simulink model "Adjustedtransfer"  (R2022a)
settings: Solver=VariableStepAuto  StartTime=0.0  StopTime=1e7  RelTol=1e-3
undefined symbols (not defined in the file): denAdjdelay, denAdjZdelay, numAdjdelay, numAdjZdelay, sigbuilder_block
libraries: cstblocks x30, slpidlib x17, slctrlblks x2
(part 1 of 2)
settings Model: Creator=emiel  LastModifiedBy=emiel
settings SolverCC: ZeroCrossAlgorithm=Adaptive
settings DebuggingCC: IgnoredZcDiagnostic=none

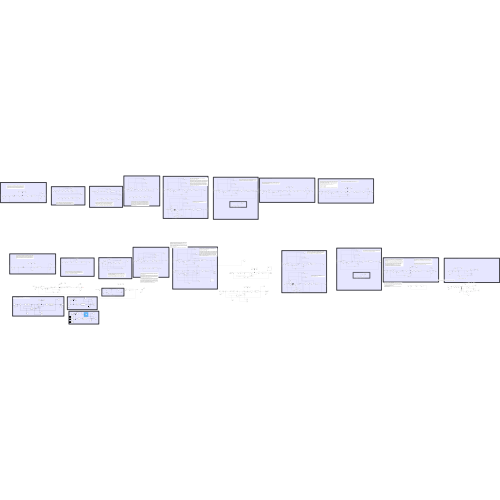
[thumbnail: Simulink's stored preview of the top-level diagram]
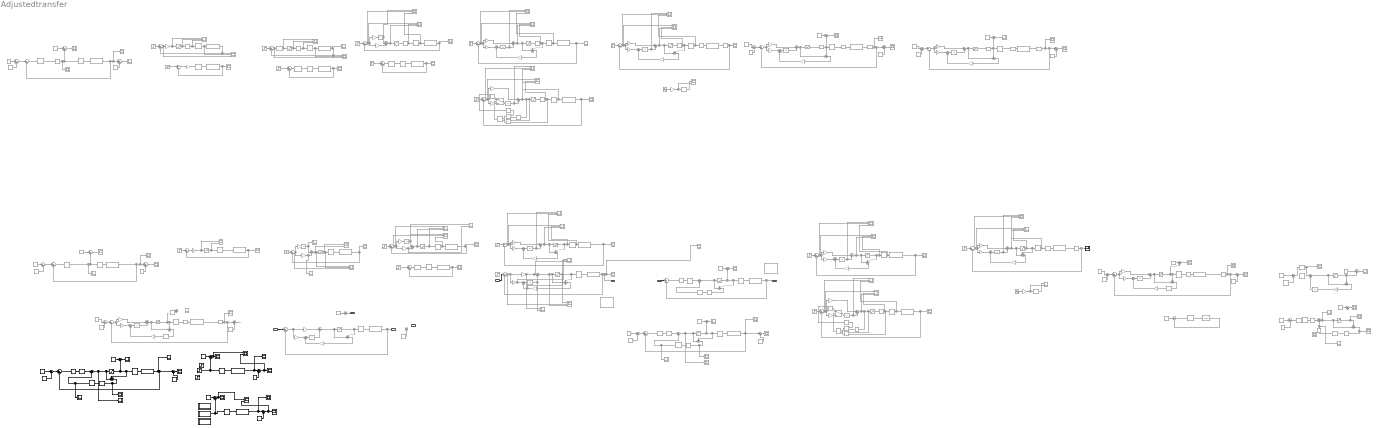
== system Adjustedtransfer ==
  note: sample tijd = 172800 ( 2 dagen) Ki en Kt = 0 en dan ziegler, Kcr = 2,31 Pcr = 347630s
      | --> Kp =  1,03, Ki = 0,00000359 en Kt = 0,00189
  note: Advise mode, een keer -0.0247
  note: Advise mode discrete controller
  note: Controller
  note: Dus als Tfruitref = -1,75 dan zijn we 56000s op -2 --> dit gebruiken als drempel voor max tijd op -2. En als we Tfruitref op -1 dan is het 7800s,
      |
      | Dus een andere vraag is "hoelang moet het groter zijn dan -2 eerdat we zeggen dat we safe zijn? Want als we zeggen, vanaf de eerste keer dat ge boven -2 zit dan kan het door fluctuaties ofzo dat ge ja toch nie oke zit.
      | 	Ge kunt beter teveel dan te weinig pakken hier.
      | Pak dat we 1800s pakken das dan 30 min, dan kunnen we wel veronderstellen dat het wel hoger dan -2 zal blijven
  note: Hier moet dan ook met discrete I controller
  note: Hier moet eigenlijk nog een schema tussen waar ik alles vervang door discrete PI controller, discrete I controller ipv die hold en ook al in de structuur die werkt voor de PLC
  note: Nog zeker eens uitzoeken wat de "responsiviteit" van een koelcel bepaald. En aangeven dat wss het opwarmen een andere snelheid heeft dan het afkoelen, en daardoor is een transferfunctie niet de optimale keuze eigelijk. Dus zou ge in dat geval non lineair moeten gaan. Maar das ja intens ma dat wel aanhalen als ja "issue"
  note: Als we naar Ts kijken zien we dan dat we 8u <-1,5 zitten. Wat opzich nog oke is. qua piekbelaasting. We zien wel dat, dde settling Ts kleiner is dan -1,025 is, da is nie veel verschil met -1 dus in de echte situatie gaan we waarchijnlijk dan nog niet op erorr = 0 zijn. Maar daarvoor dient de I actie uiteindelijk die er dan voor gaat zorgen dat da toch = 0 wodt.
  note: Dus net zeiden we de I actie wat leger voor onstabiliteit op te heffen en de P actie wat lager voor de vibraties/oscilaties op het einde. Dus we doen dan I op 0.000136 en Kt op wortel(0.000136). En we zullen dan Kp blijven verlagen vanaf 33,4 tot we een decent resultaat hebben. En vanaf Kp = 11 en Ki = 0.000136 is het goed stabiel, hebben een beetje overshoot en op het begin war vreemd maar oke nog.
      |
      | Maar als we naar U kijken zien we dat deze van +2 naar -1 gaat en das nie chill, willen liefst dat U gewoon + wordt en dan geleidelijk daalt. En we zien dat de I actie in het begin heel negatief is, dus dat wil zeggen dat Kt dan een grote invloed heeft. Dus oftewel zullen we Ki verlagen oftewel Kt of allebei.
      |
      | Als we naar de anti windup kijken zien we dat deze vooral in het begin moet werken
  note: Als we de waarde Kp en de Ki toepassen zien we dat we in beide gevallen (met en zonder satur) een onstabiel systeem hebben met veel oscilaties. Vreemd aangezien met enkel de P actie het net wel best stabiel was, dus dat wil dan zeggen dat het toevoegen van de I actie voor onstabiliteiten zorgt.
      |
      | En juist ja als we deze verlagen naar 0.000136 of nog eens /10 is het praktisch giga stabiel. Met wel een beetje oscilaties. Maar laten we toch hier eens dieper op ingaan.
  note: Eens bekijken hoelan we dan onder de -1,5 zitten want das wel lage T. exact tot 1e05 dan zitten we terug op -1,5. dus da is dan 1e05*0,8/3600 = 22u13min, da is niet kort dat is wel lang maar bij inkoelen doen ze soms 2 dagen @-2 dus het is niet onmogelijk
  note: We zien dat de P actie in het begin heel negatief is en de I actie cava positief en dan erna is de P actie cava positief en de I cava negatief, waardoor U (de som) positief wordt. Maar we willen juist een negatieve U, dus proberen om de Kp te verlagen 7,74-->5 creëren nog meer overshoot dus miss 7,74 --> 10 nu hebben we inderdaad minder overshoot als we naar Kp = 15 gaan dan is het wel mooi eigelijk
      |
      | Ongeveer idem effect hebben we als we I actie van ....e-05 naar ....e-07 (Kp = 7,74), maar dan gaat uw settling time giga toenemen. dus das ook nie chill.
      |
      | conclu Kp = 15 en Ki en Kt idem
      |
      | Kt veranderen --> instabiliteiten
      |
      | ma tegenover welke kost moeten ook miss eens kijken naar hoelang we dan op -2 zitten.
  note: Tfruit real implementeren --> terug naar het tweaken
  note: Template control schema
  note: testen van de ZOH functie
  note: Discretiseren sws ZOH willen dat de Tset en Tfruit constant blijft totdat we nieuwe T hebben. En omdat ons systeem zo traag is dan boeit da eigenlijk echt nie die discretisatie, als we ZOH op 1 zetten (0,8s) dan is het al zeker snel genoeg en pieter zegt 5ms is de cycle tijd dus zeker oke. Onze PC is eigenlijk sneller dan het systeem.
  note: Dus als we Kp = 7.74 en Ki = ....e-05 en dan Kt = wortel(...e-05) dan gaan we gekke oscilaties hebben. Maar als ik dan Kt/10 doe dan heb ik een perfect signaal.
      | Nog wel uitzoeken hoezo dat daardoor komt.µ
      |
      | Kp = 7.74, Ki= ....e-05, Kt = .....0.0045
      | Dus we zien dat de I en de P actie veel oscilaties hebben, (we zien ook dat voor saturatie en na saturatie idem is). Opmerkelijk is, is dat de P actie bena het spiegelbeeld is van de I actie, waardoor de som van de twee (de U praktisch) veel minder oscilaties hebben. We zien ook dat de I actie in het begin negatief is en dan op het einde meer positief, wat wil zeggen dat er in het begin veel saturatie optreedt en dus in het begin Kt veel moet werken. Maar in het begin willen we juist een positieve U, dus de I actie gaat eigelijk de foute kant op in het begin (doordat er saturatie is) Dus laten we dan Kt wat verlagen waardoor we de I actie in het begin minder negatief gaan maken. --> Kt = 0.00045
      | --> solved --> terugkoppelen naar de vereisten. en ook checken van step van 0-->-1 want das dalen van T en van 0-->1 is stijgen van T
  note: Implementeren van Anti-windup
  note: Simulatie van clamp wilt nie runnen en PID blok houdt geen rekening
      | met rate saturatie. Dus moeten sws handmatig doen
      | maar back caluclation is zo mooi
  note: Bewijzen dat Anti windup nodig is.
  note: Als we de Kp = 0 nemen en de Ki = ....e-07 dan zien we duidelijk dat er anti windup optreedt. Dus dit moeten we sws implementeren. We kunnen discusiëren dat als we de I actie klein genoeg nemen en de Kp niet te groot we een stabiel systeem hebben zonder dat er anti windup nodig is. Maar ten eerste ben ik niet content met dat laatste systeem, de Ess is idd = 0 maar er zijn wel wat oscilaties en overshoot en das nie chill. Ten tweede hebben we hier 1 specifieke koelcel gemodelleert. Als we een andere koelcel nemen bijvoorbeeld en daar zal er wel wind up optreden zijn we in de problemen. Ten derde de totale command is blokkerig, opeens opwarmen dan afkoelene etc. Dus we gaan eens Anti-windup implementeren
  note: Juiste Kp en Ki vinden om stabiel systeem te hebben met saturatie
  note: Als we de waarde van hierlangs toepassen dan zien we dat we een zeer stabiel systeem hebben als we geen saturatie toepassen maar een heel onstabiel als we dat wel doen. De gain is niet te hoog, laten we eens uitproberen wat het verhogen/verlagen van de I actie en de Kp als invloed heeft. Verlagen/ verhogen Kp --> (3,10,15,30) nog altijd zeer onstabiel. Verhogen Ki -->(...e-01 en ....e-03) nog altijd zeer onstabiel. Maar verlagen --> ....e-07 opeens enorm stabiel. Dus dat wil zeggen dat de I actie voor onstabiliteit zorgt.
      |
      | Hoe komt dit? --> groote I actie bekijken in alle gevallen, wss gaat er wind up optreden.
  note: Stap 1: Saturatie toevoegen.
  note: Voor deze loop was de Kcr = 73.4, maar als we de saturatie meegeven, zie hierboven zien we eigenlijk dat we op een veel lagere Kcr naar randstabiel gaan, namenlijk op 17.2 met een Pcr = 458009. Dus als we daarmee dan Ziegler nicholas toepassen krijgen we Kp = 7.74 en Ti = 3.8167e05 --> Ki = 2.0279e-05. Eens kijken wat dat geeft voor stabiliteit zonder dat we saturatie toepassen en zonder dat we anti windup toepassen?
  note: Dus dit is ons standaard model, We hebben telkens de deltaT en de deltaS gemodelleert. Dus we gaan dat ook zo in het model steken. Dus voordat we kunnen beginnen aan de PI regeling moeten we eigelijk 1 ding sws doen en liefst 2. Ten eerste moeten we de Tfruit0 en de Tset0 opmeten dat moet =! moeilijk. Gewoon de koelcel eerst opzetten en dan kijken wat het is. En dan liefst ook een step response doen en dan de parameters per koelcel bepalen voor de plant tf, maar ja als we ervan uitgaan dat da beetje oke is overal cava
  note: Discretiseren
  note: Gaan nu eigelijk terug de fruit en de set temperatuur eraan koppelen. En we zien eigenlijk dat we toch 0,1 graden undershoot hebben als we -1 fruit T willen, dus da is wel nie zo nice. Dus we gaan terug dit huidig systeem moeten analyseren om te kijken of we toch geen parameters moeten tweaken
  note: terug naar het tweaken -->
  note: Template control schema
  note: Discretiseren sws ZOH willen dat de Tset en Tfruit constant blijft totdat we nieuwe T hebben. En omdat ons systeem zo traag is dan boeit da eigenlijk echt nie die discretisatie, als we ZOH op 1s zetten dan is het al zeker snel genoeg en pieter zegt 5ms is de cycle tijd dus zeker oke. Onze PC is eigenlijk sneller dan het systeem.
  note: Implementeren van Anti-windup
  note: Bewijzen dat Anti windup nodig is.
  note: Dus als we Kp = 7.74 en Ki = ....e-05 en dan Kt = wortel(...e-05) dan gaan we gekke oscilaties hebben. Maar als ik dan Kt/10 doe dan heb ik een perfect signaal.
      | Nog wel uitzoeken hoezo dat daardoor komt.µ
      |
      | Kp = 7.74, Ki= ....e-05, Kt = .....0.0045
      | Dus we zien dat de I en de P actie veel oscilaties hebben, (we zien ook dat voor saturatie en na saturatie idem is). Opmerkelijk is, is dat de P actie bena het spiegelbeeld is van de I actie, waardoor de som van de twee (de U praktisch) veel minder oscilaties hebben. We zien ook dat de I actie in het begin negatief is en dan op het einde meer positief, wat wil zeggen dat er in het begin veel saturatie optreedt en dus in het begin Kt veel moet werken. Maar in het begin willen we juist een positieve U, dus de I actie gaat eigelijk de foute kant op in het begin (doordat er saturatie is) Dus laten we dan Kt wat verlagen waardoor we de I actie in het begin minder negatief gaan maken. --> Kt = 0.00045
      | --> solved --> terugkoppelen naar de vereisten. en ook checken van step van 0-->-1 want das dalen van T en van 0-->1 is stijgen van T
  note: Als we de Kp = 33.84 nemen en de Ki = 0.00136 dan zien we dat het systeem onstabiel is en duidelijk dat er anti windup optreedt. De I actie is gewoon giga in vergelijking met de error en de P actie. De I actie is ook max als de P actie 0 is, dus als de error 0 is. Dus anti-windup implementeren.
      |
      | Als we Ki = 0.000136 zien we dat het inderdaad stabieler maar. I actie oscileert wel al niet meer wat goed is, wat wil zeggen dat er eigenlijk geen anti windup nodig is. Dus delta T heef wel wat oscilaties --> U ook --> P ook --> error ook. Dus enkel de P actie heeft wat oscilaties, als we deze nu verlagen naar 12 of 15 hebben we minder kleine oscilaties maar meer grote/overshoot terug dus dat is het ook niet.
      |
      |  We kunnen discusiëren dat als we de I actie klein genoeg nemen en de Kp niet te groot we een stabiel systeem hebben zonder dat er anti windup nodig is. Maar ten eerste ben ik niet content met dat laatste systeem, de Ess is idd = 0 maar er zijn wel wat oscilaties en overshoot en das nie chill. Ten tweede hebben we hier 1 specifieke koelcel gemodelleert. Als we een andere koelcel nemen bijvoorbeeld en daar zal er wel wind up optreden zijn we in de problemen. Ten derde de totale command is blokkerig, opeens opwarmen dan afkoelene etc. Dus we gaan eens Anti-windup implementeren.
      |
      | Maar de P actie moet inderdaad lager om de kleine oscilaties op te lossen
  note: Tfruit real implementeren --> terug naar het tweaken
  note: Stap 1: Saturatie toevoegen.
  note: testen van de ZOH functie
  note: Dus dit is ons standaard model, We hebben telkens de deltaT en de deltaS gemodelleert. Dus we gaan dat ook zo in het model steken. Dus voordat we kunnen beginnen aan de PI regeling moeten we eigelijk 1 ding sws doen en liefst 2. Ten eerste moeten we de Tfruit0 en de Tset0 opmeten dat moet =! moeilijk. Gewoon de koelcel eerst opzetten en dan kijken wat het is. En dan liefst ook een step response doen en dan de parameters per koelcel bepalen voor de plant tf, maar ja als we ervan uitgaan dat da beetje oke is overal cava
  note: Discretiseren
  note: Gaan nu eigelijk terug de fruit en de set temperatuur eraan koppelen. En we een vreemde bult hebben in de rise, Als we dan naar de P,I en U kijken zien we dat dit door de P actie komt, dus deze nog eens verlagen van 7 naar 5 -->totaal niet de bedoeling krijgen nog gekkere bult. Verhogen naar 9 --> weinig effect op de bult, de settling time gaat alleen maar stijgen.
      |
      | I actie verhogen *10 --> bult is weg maar veel oscilatis, dus miss *5 idd minder oscilaties. *3? als we dan *2 of *3 doen hebben we terug die bult Dus miss meer oscilaties maken door I*4 en dan de Kp ook verhogen naar 10 of 15 en zien dan dat da perfect is. Hoe hoger Kp hoe groter de settling time is. Maar als ge lager dan 7 gaat met Kp dan oscilaties. Dus Kp = 12 is goeie compromis
      | xxxxxxxxxxxxxxxxxxxxxxxxxxxxxxxxxxxxxxxxxxxxxxxxxxxxxxxxxxxxxxxxxxxx
      | xxxxxxxxxxxxxxxxx--> Ki = 0,000436 en Kp = 12 en Kt = 0.01166xxxxxxxxxxx
      | xxxxxxxxxxxxxxxxxxxxxxxxxxxxxxxxxxxxxxxxxxxxxxxxxxxxxxxxxxxxxxxxxxxx
  note: Juiste Kp en Ki vinden om stabiel systeem te hebben met saturatie
  note: Voor deze loop was de Kcr = 73.4 (Kp = 33.44), maar als we de saturatie meegeven, zie hierboven zien we eigenlijk dat we op een iets hogere Kcr randstabiel gaan Kcr = 75,2 met een Pcr = 29881 . Dus als we daarmee dan Ziegler nicholas toepassen krijgen we Kp = 33.84 en --> Ki = 0.00136. Eens kijken wat dat geeft voor stabiliteit zonder dat we saturatie toepassen en zonder dat we anti windup toepassen?
  note: Oke hebben dus Kp = 11, Ki = 0.000136 en Kt = wortel(0.000136). Laten we eens kijken wat er gebeurt als we Kt/10 doen --> weinig effect op vibraties, dus terug Kt op normale en Ki/10. Systeem is nu mooi overdempt wat echt goed is. Enkle opnieuw vibraties in de P actie, nog eens verlagen dan? En dan Kp = 7 is ech wat we willen. Overdempt, U verandert niet teveel dus ideaal --> Kp = 7, Ki = 0.0000136n Kt = 0.01166
  note: Simulatie van clamp wilt nie runnen en PID blok houdt geen rekening
      | met rate saturatie. Dus moeten sws handmatig doen
      | maar back caluclation is zo mooi
  note: Implementeren van Anti-windup
  note: Schema maken om twicat te testen. Hadden net 3e6 als tijd
  note: Advise mode, -2 en dan nominaal, als we 89000s op -2°C dan zijn we op fruit T = -1.
      | Dus hebben zolang -2 gezet en dan -0.0247
  Input continious : Inport
  Input : Inport  Port=2
  Input discrete : Inport  Port=3
  -1.5°C : Subsystem  Tag=STV Subsys  LoadFcn=sigbuilder_block('load');  StartFcn=sigbuilder_block('start');  StopFcn=sigbuilder_block('stop');  ClipboardFcn=sigbuilder_block('clipboard');  mask(Sigbuilder block){tuvar=[0:10]}
      mask help: Simulink:masks:SigbuilderBlock_MD
      mask init:
      | if ~strcmp(get_param(bdroot(gcbh),'SimulationStatus'),'stopped') tuvar = sigbuilder_block('maskInit'); end
      settings: CopyFcn=sigbuilder_block('copy');  DeleteFcn=sigbuilder_block('delete');  ModelCloseFcn=sigbuilder_block('modelClose');  PreSaveFcn=sigbuilder_block('preSave');  PauseFcn=sigbuilder_block('pause');  ContinueFcn=sigbuilder_block('continue');  NameChangeFcn=sigbuilder_block('namechange');  OpenFcn=sigbuilder_block('open',[5.5 30 949 418 ]);  CloseFcn=sigbuilder_block('close');
      mask Display: plot(0, 0, 100, 100,[2, 2, 32, 32, 2], [68, 8, 8, 68, 68],[32, 2], [38, 38], [32, 19, 2],[53, 60, 44], [32, 17, 17, 2],[16, 16, 31, 31]);txt = getActiveGroup(gcbh);text(2, 100, txt,'verticalAlignment', 'top');
  -1.75°C1 : Subsystem  Tag=STV Subsys  LoadFcn=sigbuilder_block('load');  StartFcn=sigbuilder_block('start');  StopFcn=sigbuilder_block('stop');  ClipboardFcn=sigbuilder_block('clipboard');  mask(Sigbuilder block){tuvar=[0:10]}
      mask help: Simulink:masks:SigbuilderBlock_MD
      mask init:
      | if ~strcmp(get_param(bdroot(gcbh),'SimulationStatus'),'stopped') tuvar = sigbuilder_block('maskInit'); end
      settings: CopyFcn=sigbuilder_block('copy');  DeleteFcn=sigbuilder_block('delete');  ModelCloseFcn=sigbuilder_block('modelClose');  PreSaveFcn=sigbuilder_block('preSave');  PauseFcn=sigbuilder_block('pause');  ContinueFcn=sigbuilder_block('continue');  NameChangeFcn=sigbuilder_block('namechange');  OpenFcn=sigbuilder_block('open',[5.5 30 949 418 ]);  CloseFcn=sigbuilder_block('close');
      mask Display: plot(0, 0, 100, 100,[2, 2, 32, 32, 2], [68, 8, 8, 68, 68],[32, 2], [38, 38], [32, 19, 2],[53, 60, 44], [32, 17, 17, 2],[16, 16, 31, 31]);txt = getActiveGroup(gcbh);text(2, 100, txt,'verticalAlignment', 'top');
  -2°C : Subsystem  Tag=STV Subsys  LoadFcn=sigbuilder_block('load');  StartFcn=sigbuilder_block('start');  StopFcn=sigbuilder_block('stop');  ClipboardFcn=sigbuilder_block('clipboard');  mask(Sigbuilder block){tuvar=[0:10]}
      mask help: Simulink:masks:SigbuilderBlock_MD
      mask init:
      | if ~strcmp(get_param(bdroot(gcbh),'SimulationStatus'),'stopped') tuvar = sigbuilder_block('maskInit'); end
      settings: CopyFcn=sigbuilder_block('copy');  DeleteFcn=sigbuilder_block('delete');  ModelCloseFcn=sigbuilder_block('modelClose');  PreSaveFcn=sigbuilder_block('preSave');  PauseFcn=sigbuilder_block('pause');  ContinueFcn=sigbuilder_block('continue');  NameChangeFcn=sigbuilder_block('namechange');  OpenFcn=sigbuilder_block('open',[1811 5 949 418 ]);  CloseFcn=sigbuilder_block('close');
      mask Display: plot(0, 0, 100, 100,[2, 2, 32, 32, 2], [68, 8, 8, 68, 68],[32, 2], [38, 38], [32, 19, 2],[53, 60, 44], [32, 17, 17, 2],[16, 16, 31, 31]);txt = getActiveGroup(gcbh);text(2, 100, txt,'verticalAlignment', 'top');
  AND : Logic  Commented=on  IconShape=distinctive  AllPortsSameDT=off  OutDataTypeStr=boolean
  AND2 : Logic  Commented=on  IconShape=distinctive  AllPortsSameDT=off  OutDataTypeStr=boolean
  Anti windup video 2 I actie{,1..6} (7 alike) : Scope  Commented=on  NumInputPorts=3
  Anti windup video 2 I actie clamp : Scope  Commented=on  NumInputPorts=3
  Anti windup video 2 I actie clamp2 : Scope  Commented=on  NumInputPorts=3
  Anti windup video totale command{,1..5,7..9} (9 alike) : Scope  Commented=on  NumInputPorts=3
  Anti-windup Kt : slpidlib/PID Controller  Commented=on  Controller=I  Form=Parallel  TimeDomain=Continuous-time  UseExternalTs=off  SampleTime=-1  IntegratorMethod=Forward Euler  FilterMethod=Forward Euler  ControllerParametersSource=internal  P=1  I=0.000368  UseKiTs=off  D=0  N=100  UseFilter=on  TunerSelectOption=Transfer Function Based (PID Tuner App)  InitialConditionSource=internal  InitialConditionForIntegrator=0  InitialConditionForFilter=0  DifferentiatorICPrevScaledInput=0  ExternalReset=none  TrackingMode=off  Kt=1  LimitOutput=off  SatLimitsSource=internal  UpperSaturationLimit=inf  LowerSaturationLimit=-inf  LinearizeAsGain=off  AntiWindupMode=none  Kb=1  POutMin=[]  POutMax=[]  IOutMin=[]  IOutMax=[]  DOutMin=[]  DOutMax=[]  NOutMin=[]  NOutMax=[]  SumOutMin=[]  SumOutMax=[]  SaturationOutMin=[]  SaturationOutMax=[]  PParamMin=[]  PParamMax=[]  IParamMin=[]  IParamMax=[]  DParamMin=[]  DParamMax=[]  NParamMin=[]  NParamMax=[]  KbParamMin=[]  KbParamMax=[]  KtParamMin=[]  KtParamMax=[]  KbOutMin=[]  KbOutMax=[]  KtOutMin=[]  KtOutMax=[]  IntegratorOutMin=[]  IntegratorOutMax=[]  FilterOutMin=[]  FilterOutMax=[]  SumI1OutMin=[]  SumI1OutMax=[]  SumI2OutMin=[]  SumI2OutMax=[]  SumI3OutMin=[]  SumI3OutMax=[]  SumI4OutMin=[]  SumI4OutMax=[]  SumDOutMin=[]  SumDOutMax=[]  DifferentiatorOutMin=[]  DifferentiatorOutMax=[]  FilterDiffOutCoefMin=[]  FilterDiffOutCoefMax=[]  ReciprocalOutMin=[]  ReciprocalOutMax=[]  SumDenOutMin=[]  SumDenOutMax=[]  SumNumOutMin=[]  SumNumOutMax=[]  DivideOutMin=[]  DivideOutMax=[]  UdiffTsProdOutMin=[]  UdiffTsProdOutMax=[]  NTsProdOutMin=[]  NTsProdOutMax=[]  UintegralTsProdOutMin=[]  UintegralTsProdOutMax=[]  UngainTsProdOutMin=[]  UngainTsProdOutMax=[]  IntegratorContinuousStateAttributes=''  IntegratorStateMustResolveToSignalObject=off  IntegratorRTWStateStorageClass=Auto  FilterContinuousStateAttributes=''  FilterStateMustResolveToSignalObject=off  FilterRTWStateStorageClass=Auto  ParallelPVariant=Disabled  IdealPVariant=Disabled  IVariant=InternalParameters  DVariant=Disabled  IntegratorVariant=Continuous  SatVariant=Disabled  AWVariant=Passthrough  PCopyVariant=Disabled  TRVariant=Disabled  FdbkBlocksVariant=Forward  IdealPFdbkVariant=Disabled  SatFdbkVariant=Disabled  DerivativeFilterVariant=Disabled  NVariant=Disabled  NCopyVariant=Disabled_SignalSpec  FilterICVariant=Disabled  IntegratorICVariant=InternalICs  ExternalResetVariant=Disabled  TRSumVariant=Passthrough  SumFdbkVariant=Disabled  SumVariant=Passthrough_I  TsampFilterVariant=InternalTs  TsampNgainVariant=Passthrough  TsampIntegralVariant=Passthrough  ExternalSaturationOutDataTypeStr=Inherit: Same as second input  aMode=0
  "Anti-windup Kt    " : slpidlib/PID Controller  Commented=on  Controller=I  Form=Parallel  TimeDomain=Continuous-time  UseExternalTs=off  SampleTime=-1  IntegratorMethod=Forward Euler  FilterMethod=Forward Euler  ControllerParametersSource=internal  P=1  I=0.0368  UseKiTs=off  D=0  N=100  UseFilter=on  TunerSelectOption=Transfer Function Based (PID Tuner App)  InitialConditionSource=internal  InitialConditionForIntegrator=0  InitialConditionForFilter=0  DifferentiatorICPrevScaledInput=0  ExternalReset=none  TrackingMode=off  Kt=1  LimitOutput=off  SatLimitsSource=internal  UpperSaturationLimit=inf  LowerSaturationLimit=-inf  LinearizeAsGain=off  AntiWindupMode=none  Kb=1  POutMin=[]  POutMax=[]  IOutMin=[]  IOutMax=[]  DOutMin=[]  DOutMax=[]  NOutMin=[]  NOutMax=[]  SumOutMin=[]  SumOutMax=[]  SaturationOutMin=[]  SaturationOutMax=[]  PParamMin=[]  PParamMax=[]  IParamMin=[]  IParamMax=[]  DParamMin=[]  DParamMax=[]  NParamMin=[]  NParamMax=[]  KbParamMin=[]  KbParamMax=[]  KtParamMin=[]  KtParamMax=[]  KbOutMin=[]  KbOutMax=[]  KtOutMin=[]  KtOutMax=[]  IntegratorOutMin=[]  IntegratorOutMax=[]  FilterOutMin=[]  FilterOutMax=[]  SumI1OutMin=[]  SumI1OutMax=[]  SumI2OutMin=[]  SumI2OutMax=[]  SumI3OutMin=[]  SumI3OutMax=[]  SumI4OutMin=[]  SumI4OutMax=[]  SumDOutMin=[]  SumDOutMax=[]  DifferentiatorOutMin=[]  DifferentiatorOutMax=[]  FilterDiffOutCoefMin=[]  FilterDiffOutCoefMax=[]  ReciprocalOutMin=[]  ReciprocalOutMax=[]  SumDenOutMin=[]  SumDenOutMax=[]  SumNumOutMin=[]  SumNumOutMax=[]  DivideOutMin=[]  DivideOutMax=[]  UdiffTsProdOutMin=[]  UdiffTsProdOutMax=[]  NTsProdOutMin=[]  NTsProdOutMax=[]  UintegralTsProdOutMin=[]  UintegralTsProdOutMax=[]  UngainTsProdOutMin=[]  UngainTsProdOutMax=[]  IntegratorContinuousStateAttributes=''  IntegratorStateMustResolveToSignalObject=off  IntegratorRTWStateStorageClass=Auto  FilterContinuousStateAttributes=''  FilterStateMustResolveToSignalObject=off  FilterRTWStateStorageClass=Auto  ParallelPVariant=Disabled  IdealPVariant=Disabled  IVariant=InternalParameters  DVariant=Disabled  IntegratorVariant=Continuous  SatVariant=Disabled  AWVariant=Passthrough  PCopyVariant=Disabled  TRVariant=Disabled  FdbkBlocksVariant=Forward  IdealPFdbkVariant=Disabled  SatFdbkVariant=Disabled  DerivativeFilterVariant=Disabled  NVariant=Disabled  NCopyVariant=Disabled_SignalSpec  FilterICVariant=Disabled  IntegratorICVariant=InternalICs  ExternalResetVariant=Disabled  TRSumVariant=Passthrough  SumFdbkVariant=Disabled  SumVariant=Passthrough_I  TsampFilterVariant=InternalTs  TsampNgainVariant=Passthrough  TsampIntegralVariant=Passthrough  ExternalSaturationOutDataTypeStr=Inherit: Same as second input  aMode=0
  Anti-windup Kt1 : slpidlib/PID Controller  Commented=on  Controller=I  Form=Parallel  TimeDomain=Continuous-time  UseExternalTs=off  SampleTime=-1  IntegratorMethod=Forward Euler  FilterMethod=Forward Euler  ControllerParametersSource=internal  P=1  I=0.000368  UseKiTs=off  D=0  N=100  UseFilter=on  TunerSelectOption=Transfer Function Based (PID Tuner App)  InitialConditionSource=internal  InitialConditionForIntegrator=0  InitialConditionForFilter=0  DifferentiatorICPrevScaledInput=0  ExternalReset=none  TrackingMode=off  Kt=1  LimitOutput=off  SatLimitsSource=internal  UpperSaturationLimit=inf  LowerSaturationLimit=-inf  LinearizeAsGain=off  AntiWindupMode=none  Kb=1  POutMin=[]  POutMax=[]  IOutMin=[]  IOutMax=[]  DOutMin=[]  DOutMax=[]  NOutMin=[]  NOutMax=[]  SumOutMin=[]  SumOutMax=[]  SaturationOutMin=[]  SaturationOutMax=[]  PParamMin=[]  PParamMax=[]  IParamMin=[]  IParamMax=[]  DParamMin=[]  DParamMax=[]  NParamMin=[]  NParamMax=[]  KbParamMin=[]  KbParamMax=[]  KtParamMin=[]  KtParamMax=[]  KbOutMin=[]  KbOutMax=[]  KtOutMin=[]  KtOutMax=[]  IntegratorOutMin=[]  IntegratorOutMax=[]  FilterOutMin=[]  FilterOutMax=[]  SumI1OutMin=[]  SumI1OutMax=[]  SumI2OutMin=[]  SumI2OutMax=[]  SumI3OutMin=[]  SumI3OutMax=[]  SumI4OutMin=[]  SumI4OutMax=[]  SumDOutMin=[]  SumDOutMax=[]  DifferentiatorOutMin=[]  DifferentiatorOutMax=[]  FilterDiffOutCoefMin=[]  FilterDiffOutCoefMax=[]  ReciprocalOutMin=[]  ReciprocalOutMax=[]  SumDenOutMin=[]  SumDenOutMax=[]  SumNumOutMin=[]  SumNumOutMax=[]  DivideOutMin=[]  DivideOutMax=[]  UdiffTsProdOutMin=[]  UdiffTsProdOutMax=[]  NTsProdOutMin=[]  NTsProdOutMax=[]  UintegralTsProdOutMin=[]  UintegralTsProdOutMax=[]  UngainTsProdOutMin=[]  UngainTsProdOutMax=[]  IntegratorContinuousStateAttributes=''  IntegratorStateMustResolveToSignalObject=off  IntegratorRTWStateStorageClass=Auto  FilterContinuousStateAttributes=''  FilterStateMustResolveToSignalObject=off  FilterRTWStateStorageClass=Auto  ParallelPVariant=Disabled  IdealPVariant=Disabled  IVariant=InternalParameters  DVariant=Disabled  IntegratorVariant=Continuous  SatVariant=Disabled  AWVariant=Passthrough  PCopyVariant=Disabled  TRVariant=Disabled  FdbkBlocksVariant=Forward  IdealPFdbkVariant=Disabled  SatFdbkVariant=Disabled  DerivativeFilterVariant=Disabled  NVariant=Disabled  NCopyVariant=Disabled_SignalSpec  FilterICVariant=Disabled  IntegratorICVariant=InternalICs  ExternalResetVariant=Disabled  TRSumVariant=Passthrough  SumFdbkVariant=Disabled  SumVariant=Passthrough_I  TsampFilterVariant=InternalTs  TsampNgainVariant=Passthrough  TsampIntegralVariant=Passthrough  ExternalSaturationOutDataTypeStr=Inherit: Same as second input  aMode=0
  Anti-windup Kt2 : slpidlib/PID Controller  Controller=I  Form=Parallel  TimeDomain=Continuous-time  UseExternalTs=off  SampleTime=-1  IntegratorMethod=Forward Euler  FilterMethod=Forward Euler  ControllerParametersSource=internal  P=1  I=0.0435  UseKiTs=off  D=0  N=100  UseFilter=on  TunerSelectOption=Transfer Function Based (PID Tuner App)  InitialConditionSource=internal  InitialConditionForIntegrator=0  InitialConditionForFilter=0  DifferentiatorICPrevScaledInput=0  ExternalReset=none  TrackingMode=off  Kt=1  LimitOutput=off  SatLimitsSource=internal  UpperSaturationLimit=inf  LowerSaturationLimit=-inf  LinearizeAsGain=off  AntiWindupMode=none  Kb=1  POutMin=[]  POutMax=[]  IOutMin=[]  IOutMax=[]  DOutMin=[]  DOutMax=[]  NOutMin=[]  NOutMax=[]  SumOutMin=[]  SumOutMax=[]  SaturationOutMin=[]  SaturationOutMax=[]  PParamMin=[]  PParamMax=[]  IParamMin=[]  IParamMax=[]  DParamMin=[]  DParamMax=[]  NParamMin=[]  NParamMax=[]  KbParamMin=[]  KbParamMax=[]  KtParamMin=[]  KtParamMax=[]  KbOutMin=[]  KbOutMax=[]  KtOutMin=[]  KtOutMax=[]  IntegratorOutMin=[]  IntegratorOutMax=[]  FilterOutMin=[]  FilterOutMax=[]  SumI1OutMin=[]  SumI1OutMax=[]  SumI2OutMin=[]  SumI2OutMax=[]  SumI3OutMin=[]  SumI3OutMax=[]  SumI4OutMin=[]  SumI4OutMax=[]  SumDOutMin=[]  SumDOutMax=[]  DifferentiatorOutMin=[]  DifferentiatorOutMax=[]  FilterDiffOutCoefMin=[]  FilterDiffOutCoefMax=[]  ReciprocalOutMin=[]  ReciprocalOutMax=[]  SumDenOutMin=[]  SumDenOutMax=[]  SumNumOutMin=[]  SumNumOutMax=[]  DivideOutMin=[]  DivideOutMax=[]  UdiffTsProdOutMin=[]  UdiffTsProdOutMax=[]  NTsProdOutMin=[]  NTsProdOutMax=[]  UintegralTsProdOutMin=[]  UintegralTsProdOutMax=[]  UngainTsProdOutMin=[]  UngainTsProdOutMax=[]  IntegratorContinuousStateAttributes=''  IntegratorStateMustResolveToSignalObject=off  IntegratorRTWStateStorageClass=Auto  FilterContinuousStateAttributes=''  FilterStateMustResolveToSignalObject=off  FilterRTWStateStorageClass=Auto  ParallelPVariant=Disabled  IdealPVariant=Disabled  IVariant=InternalParameters  DVariant=Disabled  IntegratorVariant=Continuous  SatVariant=Disabled  AWVariant=Passthrough  PCopyVariant=Disabled  TRVariant=Disabled  FdbkBlocksVariant=Forward  IdealPFdbkVariant=Disabled  SatFdbkVariant=Disabled  DerivativeFilterVariant=Disabled  NVariant=Disabled  NCopyVariant=Disabled_SignalSpec  FilterICVariant=Disabled  IntegratorICVariant=InternalICs  ExternalResetVariant=Disabled  TRSumVariant=Passthrough  SumFdbkVariant=Disabled  SumVariant=Passthrough_I  TsampFilterVariant=InternalTs  TsampNgainVariant=Passthrough  TsampIntegralVariant=Passthrough  ExternalSaturationOutDataTypeStr=Inherit: Same as second input  aMode=0
  Bias1 : Constant  Commented=on  Value=-1
  Bias2 : Constant  Commented=on  Value=-1
  Bode Plot : slctrlblks/Model Verification/Check Bode  Characteristics  Commented=on  InstantiateOnLoad=on  SaveOperatingPoints=off  LinearizationIOs={'/Plant discrete', 1, 'out', 'on', '';'/Input discrete', 1, 'in', 'on', ''}  LinearizeAt=SnapshotTimes  SnapshotTimes=[0]  TriggerType=rising  SampleTime=auto  RateConversionMethod=zoh  PreWarpFreq=10  UseExactDelayModel=off  UseFullBlockNameLabels=off  UseBusSignalLabels=off  enabled=on  stopWhenAssertionFail=off  export=off  ViewDlgPos=[3.66666666666667 232.333333333333 538.666666666667 390]  OpenViewOnLoad=off  LaunchViewOnOpen=off  FrequencyUnits=rad/s  MagnitudeUnits=dB  PhaseUnits=deg  TimeUnits=seconds  EnableUpperBound=off  UpperBoundFrequencies=[]  UpperBoundMagnitudes=[]  EnableLowerBound=off  LowerBoundFrequencies=[]  LowerBoundMagnitudes=[]
  Bode Plot1 : slctrlblks/Model Verification/Check Bode  Characteristics  Commented=on  InstantiateOnLoad=on  SaveOperatingPoints=off  LinearizationIOs={'/Plant continious', 1, 'out', 'on', '';'/Input continious', 1, 'in', 'on', ''}  LinearizeAt=SnapshotTimes  SnapshotTimes=[0]  TriggerType=rising  SampleTime=auto  RateConversionMethod=zoh  PreWarpFreq=10  UseExactDelayModel=off  UseFullBlockNameLabels=off  UseBusSignalLabels=off  enabled=on  stopWhenAssertionFail=off  export=off  ViewDlgPos=[2151 -28.3333333333333 733.333333333333 528]  OpenViewOnLoad=off  LaunchViewOnOpen=off  FrequencyUnits=rad/s  MagnitudeUnits=dB  PhaseUnits=deg  TimeUnits=seconds  EnableUpperBound=off  UpperBoundFrequencies=[]  UpperBoundMagnitudes=[]  EnableLowerBound=off  LowerBoundFrequencies=[]  LowerBoundMagnitudes=[]
      settings: SaveToWorkspace=on  SaveName=sys2
  Constant{1..4} (4 alike) : Constant  Commented=on  Value=-0.75
  Constant5 : Constant  Commented=on  Value=0
  Constant6 : Constant  Commented=on  Value=-1
  Constant8 : Constant  Commented=on  Value=-1
  Constant9 : Constant  Commented=on  Value=0
  Continious model{,1..3} (4 alike) : Scope  Commented=on
  Delta S : Scope  Commented=on
  Delta S1 : Scope  Commented=on
  Discrete PID Controller : slpidlib/PID Controller  Commented=on  Controller=PI  Form=Parallel  TimeDomain=Discrete-time  UseExternalTs=off  SampleTime=1  IntegratorMethod=Backward Euler  FilterMethod=Backward Euler  ControllerParametersSource=internal  P=12  I=0.0000436  UseKiTs=off  D=0  N=100  UseFilter=on  TunerSelectOption=Transfer Function Based (PID Tuner App)  InitialConditionSource=internal  InitialConditionForIntegrator=0  InitialConditionForFilter=0  DifferentiatorICPrevScaledInput=0  ExternalReset=none  TrackingMode=off  Kt=1  LimitOutput=off  SatLimitsSource=internal  UpperSaturationLimit=inf  LowerSaturationLimit=-inf  LinearizeAsGain=off  AntiWindupMode=none  Kb=1  POutMin=[]  POutMax=[]  IOutMin=[]  IOutMax=[]  DOutMin=[]  DOutMax=[]  NOutMin=[]  NOutMax=[]  SumOutMin=[]  SumOutMax=[]  SaturationOutMin=[]  SaturationOutMax=[]  PParamMin=[]  PParamMax=[]  IParamMin=[]  IParamMax=[]  DParamMin=[]  DParamMax=[]  NParamMin=[]  NParamMax=[]  KbParamMin=[]  KbParamMax=[]  KtParamMin=[]  KtParamMax=[]  KbOutMin=[]  KbOutMax=[]  KtOutMin=[]  KtOutMax=[]  IntegratorOutMin=[]  IntegratorOutMax=[]  FilterOutMin=[]  FilterOutMax=[]  SumI1OutMin=[]  SumI1OutMax=[]  SumI2OutMin=[]  SumI2OutMax=[]  SumI3OutMin=[]  SumI3OutMax=[]  SumI4OutMin=[]  SumI4OutMax=[]  SumDOutMin=[]  SumDOutMax=[]  DifferentiatorOutMin=[]  DifferentiatorOutMax=[]  FilterDiffOutCoefMin=[]  FilterDiffOutCoefMax=[]  ReciprocalOutMin=[]  ReciprocalOutMax=[]  SumDenOutMin=[]  SumDenOutMax=[]  SumNumOutMin=[]  SumNumOutMax=[]  DivideOutMin=[]  DivideOutMax=[]  UdiffTsProdOutMin=[]  UdiffTsProdOutMax=[]  NTsProdOutMin=[]  NTsProdOutMax=[]  UintegralTsProdOutMin=[]  UintegralTsProdOutMax=[]  UngainTsProdOutMin=[]  UngainTsProdOutMax=[]  IntegratorContinuousStateAttributes=''  IntegratorStateMustResolveToSignalObject=off  IntegratorRTWStateStorageClass=Auto  FilterContinuousStateAttributes=''  FilterStateMustResolveToSignalObject=off  FilterRTWStateStorageClass=Auto  ParallelPVariant=InternalParameters  IdealPVariant=Disabled  IVariant=InternalParameters  DVariant=Disabled  IntegratorVariant=Discrete  SatVariant=Disabled  AWVariant=Passthrough  PCopyVariant=Disabled  TRVariant=Disabled  FdbkBlocksVariant=Forward  IdealPFdbkVariant=Disabled  SatFdbkVariant=Disabled  DerivativeFilterVariant=Disabled  NVariant=Disabled  NCopyVariant=Disabled_SignalSpec  FilterICVariant=Disabled  IntegratorICVariant=InternalICs  ExternalResetVariant=Disabled  TRSumVariant=Passthrough  SumFdbkVariant=Disabled  SumVariant=Sum_PI  TsampFilterVariant=InternalTs  TsampNgainVariant=Passthrough  TsampIntegralVariant=Passthrough  ExternalSaturationOutDataTypeStr=Inherit: Same as second input  aMode=0
  Discrete PID Controller1 : slpidlib/PID Controller  Commented=on  Controller=PI  Form=Parallel  TimeDomain=Continuous-time  UseExternalTs=off  SampleTime=1  IntegratorMethod=Backward Euler  FilterMethod=Forward Euler  ControllerParametersSource=internal  P=15  I=0.000136  UseKiTs=off  D=0  N=100  UseFilter=on  TunerSelectOption=Transfer Function Based (PID Tuner App)  InitialConditionSource=internal  InitialConditionForIntegrator=0  InitialConditionForFilter=0  DifferentiatorICPrevScaledInput=0  ExternalReset=none  TrackingMode=off  Kt=1  LimitOutput=off  SatLimitsSource=internal  UpperSaturationLimit=inf  LowerSaturationLimit=-inf  LinearizeAsGain=off  AntiWindupMode=none  Kb=1  POutMin=[]  POutMax=[]  IOutMin=[]  IOutMax=[]  DOutMin=[]  DOutMax=[]  NOutMin=[]  NOutMax=[]  SumOutMin=[]  SumOutMax=[]  SaturationOutMin=[]  SaturationOutMax=[]  PParamMin=[]  PParamMax=[]  IParamMin=[]  IParamMax=[]  DParamMin=[]  DParamMax=[]  NParamMin=[]  NParamMax=[]  KbParamMin=[]  KbParamMax=[]  KtParamMin=[]  KtParamMax=[]  KbOutMin=[]  KbOutMax=[]  KtOutMin=[]  KtOutMax=[]  IntegratorOutMin=[]  IntegratorOutMax=[]  FilterOutMin=[]  FilterOutMax=[]  SumI1OutMin=[]  SumI1OutMax=[]  SumI2OutMin=[]  SumI2OutMax=[]  SumI3OutMin=[]  SumI3OutMax=[]  SumI4OutMin=[]  SumI4OutMax=[]  SumDOutMin=[]  SumDOutMax=[]  DifferentiatorOutMin=[]  DifferentiatorOutMax=[]  FilterDiffOutCoefMin=[]  FilterDiffOutCoefMax=[]  ReciprocalOutMin=[]  ReciprocalOutMax=[]  SumDenOutMin=[]  SumDenOutMax=[]  SumNumOutMin=[]  SumNumOutMax=[]  DivideOutMin=[]  DivideOutMax=[]  UdiffTsProdOutMin=[]  UdiffTsProdOutMax=[]  NTsProdOutMin=[]  NTsProdOutMax=[]  UintegralTsProdOutMin=[]  UintegralTsProdOutMax=[]  UngainTsProdOutMin=[]  UngainTsProdOutMax=[]  IntegratorContinuousStateAttributes=''  IntegratorStateMustResolveToSignalObject=off  IntegratorRTWStateStorageClass=Auto  FilterContinuousStateAttributes=''  FilterStateMustResolveToSignalObject=off  FilterRTWStateStorageClass=Auto  ParallelPVariant=InternalParameters  IdealPVariant=Disabled  IVariant=InternalParameters  DVariant=Disabled  IntegratorVariant=Continuous  SatVariant=Disabled  AWVariant=Passthrough  PCopyVariant=Disabled  TRVariant=Disabled  FdbkBlocksVariant=Forward  IdealPFdbkVariant=Disabled  SatFdbkVariant=Disabled  DerivativeFilterVariant=Disabled  NVariant=Disabled  NCopyVariant=Disabled_SignalSpec  FilterICVariant=Disabled  IntegratorICVariant=InternalICs  ExternalResetVariant=Disabled  TRSumVariant=Passthrough  SumFdbkVariant=Disabled  SumVariant=Sum_PI  TsampFilterVariant=InternalTs  TsampNgainVariant=Passthrough  TsampIntegralVariant=Passthrough  ExternalSaturationOutDataTypeStr=Inherit: Same as second input  aMode=0
  Discrete PID Controller2 : slpidlib/PID Controller  Commented=on  Controller=PI  Form=Parallel  TimeDomain=Continuous-time  UseExternalTs=off  SampleTime=1  IntegratorMethod=Backward Euler  FilterMethod=Forward Euler  ControllerParametersSource=internal  P=15  I=0.0136  UseKiTs=off  D=0  N=100  UseFilter=on  TunerSelectOption=Transfer Function Based (PID Tuner App)  InitialConditionSource=internal  InitialConditionForIntegrator=0  InitialConditionForFilter=0  DifferentiatorICPrevScaledInput=0  ExternalReset=none  TrackingMode=off  Kt=1  LimitOutput=off  SatLimitsSource=internal  UpperSaturationLimit=inf  LowerSaturationLimit=-inf  LinearizeAsGain=off  AntiWindupMode=none  Kb=1  POutMin=[]  POutMax=[]  IOutMin=[]  IOutMax=[]  DOutMin=[]  DOutMax=[]  NOutMin=[]  NOutMax=[]  SumOutMin=[]  SumOutMax=[]  SaturationOutMin=[]  SaturationOutMax=[]  PParamMin=[]  PParamMax=[]  IParamMin=[]  IParamMax=[]  DParamMin=[]  DParamMax=[]  NParamMin=[]  NParamMax=[]  KbParamMin=[]  KbParamMax=[]  KtParamMin=[]  KtParamMax=[]  KbOutMin=[]  KbOutMax=[]  KtOutMin=[]  KtOutMax=[]  IntegratorOutMin=[]  IntegratorOutMax=[]  FilterOutMin=[]  FilterOutMax=[]  SumI1OutMin=[]  SumI1OutMax=[]  SumI2OutMin=[]  SumI2OutMax=[]  SumI3OutMin=[]  SumI3OutMax=[]  SumI4OutMin=[]  SumI4OutMax=[]  SumDOutMin=[]  SumDOutMax=[]  DifferentiatorOutMin=[]  DifferentiatorOutMax=[]  FilterDiffOutCoefMin=[]  FilterDiffOutCoefMax=[]  ReciprocalOutMin=[]  ReciprocalOutMax=[]  SumDenOutMin=[]  SumDenOutMax=[]  SumNumOutMin=[]  SumNumOutMax=[]  DivideOutMin=[]  DivideOutMax=[]  UdiffTsProdOutMin=[]  UdiffTsProdOutMax=[]  NTsProdOutMin=[]  NTsProdOutMax=[]  UintegralTsProdOutMin=[]  UintegralTsProdOutMax=[]  UngainTsProdOutMin=[]  UngainTsProdOutMax=[]  IntegratorContinuousStateAttributes=''  IntegratorStateMustResolveToSignalObject=off  IntegratorRTWStateStorageClass=Auto  FilterContinuousStateAttributes=''  FilterStateMustResolveToSignalObject=off  FilterRTWStateStorageClass=Auto  ParallelPVariant=InternalParameters  IdealPVariant=Disabled  IVariant=InternalParameters  DVariant=Disabled  IntegratorVariant=Continuous  SatVariant=Disabled  AWVariant=Passthrough  PCopyVariant=Disabled  TRVariant=Disabled  FdbkBlocksVariant=Forward  IdealPFdbkVariant=Disabled  SatFdbkVariant=Disabled  DerivativeFilterVariant=Disabled  NVariant=Disabled  NCopyVariant=Disabled_SignalSpec  FilterICVariant=Disabled  IntegratorICVariant=InternalICs  ExternalResetVariant=Disabled  TRSumVariant=Passthrough  SumFdbkVariant=Disabled  SumVariant=Sum_PI  TsampFilterVariant=InternalTs  TsampNgainVariant=Passthrough  TsampIntegralVariant=Passthrough  ExternalSaturationOutDataTypeStr=Inherit: Same as second input  aMode=0
  Discrete PID Controller3 : slpidlib/PID Controller  Commented=on  Controller=PI  Form=Parallel  TimeDomain=Continuous-time  UseExternalTs=off  SampleTime=1  IntegratorMethod=Backward Euler  FilterMethod=Forward Euler  ControllerParametersSource=internal  P=15  I=0.000136  UseKiTs=off  D=0  N=100  UseFilter=on  TunerSelectOption=Transfer Function Based (PID Tuner App)  InitialConditionSource=internal  InitialConditionForIntegrator=0  InitialConditionForFilter=0  DifferentiatorICPrevScaledInput=0  ExternalReset=none  TrackingMode=off  Kt=1  LimitOutput=off  SatLimitsSource=internal  UpperSaturationLimit=inf  LowerSaturationLimit=-inf  LinearizeAsGain=off  AntiWindupMode=none  Kb=1  POutMin=[]  POutMax=[]  IOutMin=[]  IOutMax=[]  DOutMin=[]  DOutMax=[]  NOutMin=[]  NOutMax=[]  SumOutMin=[]  SumOutMax=[]  SaturationOutMin=[]  SaturationOutMax=[]  PParamMin=[]  PParamMax=[]  IParamMin=[]  IParamMax=[]  DParamMin=[]  DParamMax=[]  NParamMin=[]  NParamMax=[]  KbParamMin=[]  KbParamMax=[]  KtParamMin=[]  KtParamMax=[]  KbOutMin=[]  KbOutMax=[]  KtOutMin=[]  KtOutMax=[]  IntegratorOutMin=[]  IntegratorOutMax=[]  FilterOutMin=[]  FilterOutMax=[]  SumI1OutMin=[]  SumI1OutMax=[]  SumI2OutMin=[]  SumI2OutMax=[]  SumI3OutMin=[]  SumI3OutMax=[]  SumI4OutMin=[]  SumI4OutMax=[]  SumDOutMin=[]  SumDOutMax=[]  DifferentiatorOutMin=[]  DifferentiatorOutMax=[]  FilterDiffOutCoefMin=[]  FilterDiffOutCoefMax=[]  ReciprocalOutMin=[]  ReciprocalOutMax=[]  SumDenOutMin=[]  SumDenOutMax=[]  SumNumOutMin=[]  SumNumOutMax=[]  DivideOutMin=[]  DivideOutMax=[]  UdiffTsProdOutMin=[]  UdiffTsProdOutMax=[]  NTsProdOutMin=[]  NTsProdOutMax=[]  UintegralTsProdOutMin=[]  UintegralTsProdOutMax=[]  UngainTsProdOutMin=[]  UngainTsProdOutMax=[]  IntegratorContinuousStateAttributes=''  IntegratorStateMustResolveToSignalObject=off  IntegratorRTWStateStorageClass=Auto  FilterContinuousStateAttributes=''  FilterStateMustResolveToSignalObject=off  FilterRTWStateStorageClass=Auto  ParallelPVariant=InternalParameters  IdealPVariant=Disabled  IVariant=InternalParameters  DVariant=Disabled  IntegratorVariant=Continuous  SatVariant=Disabled  AWVariant=Passthrough  PCopyVariant=Disabled  TRVariant=Disabled  FdbkBlocksVariant=Forward  IdealPFdbkVariant=Disabled  SatFdbkVariant=Disabled  DerivativeFilterVariant=Disabled  NVariant=Disabled  NCopyVariant=Disabled_SignalSpec  FilterICVariant=Disabled  IntegratorICVariant=InternalICs  ExternalResetVariant=Disabled  TRSumVariant=Passthrough  SumFdbkVariant=Disabled  SumVariant=Sum_PI  TsampFilterVariant=InternalTs  TsampNgainVariant=Passthrough  TsampIntegralVariant=Passthrough  ExternalSaturationOutDataTypeStr=Inherit: Same as second input  aMode=0
  Discrete PID Controller4 : slpidlib/PID Controller  Controller=PI  Form=Parallel  TimeDomain=Continuous-time  UseExternalTs=off  SampleTime=1  IntegratorMethod=Backward Euler  FilterMethod=Forward Euler  ControllerParametersSource=internal  P=0.5  I=0.000000359  UseKiTs=off  D=0  N=100  UseFilter=on  TunerSelectOption=Transfer Function Based (PID Tuner App)  InitialConditionSource=internal  InitialConditionForIntegrator=0  InitialConditionForFilter=0  DifferentiatorICPrevScaledInput=0  ExternalReset=none  TrackingMode=off  Kt=1  LimitOutput=off  SatLimitsSource=internal  UpperSaturationLimit=inf  LowerSaturationLimit=-inf  LinearizeAsGain=off  AntiWindupMode=none  Kb=1  POutMin=[]  POutMax=[]  IOutMin=[]  IOutMax=[]  DOutMin=[]  DOutMax=[]  NOutMin=[]  NOutMax=[]  SumOutMin=[]  SumOutMax=[]  SaturationOutMin=[]  SaturationOutMax=[]  PParamMin=[]  PParamMax=[]  IParamMin=[]  IParamMax=[]  DParamMin=[]  DParamMax=[]  NParamMin=[]  NParamMax=[]  KbParamMin=[]  KbParamMax=[]  KtParamMin=[]  KtParamMax=[]  KbOutMin=[]  KbOutMax=[]  KtOutMin=[]  KtOutMax=[]  IntegratorOutMin=[]  IntegratorOutMax=[]  FilterOutMin=[]  FilterOutMax=[]  SumI1OutMin=[]  SumI1OutMax=[]  SumI2OutMin=[]  SumI2OutMax=[]  SumI3OutMin=[]  SumI3OutMax=[]  SumI4OutMin=[]  SumI4OutMax=[]  SumDOutMin=[]  SumDOutMax=[]  DifferentiatorOutMin=[]  DifferentiatorOutMax=[]  FilterDiffOutCoefMin=[]  FilterDiffOutCoefMax=[]  ReciprocalOutMin=[]  ReciprocalOutMax=[]  SumDenOutMin=[]  SumDenOutMax=[]  SumNumOutMin=[]  SumNumOutMax=[]  DivideOutMin=[]  DivideOutMax=[]  UdiffTsProdOutMin=[]  UdiffTsProdOutMax=[]  NTsProdOutMin=[]  NTsProdOutMax=[]  UintegralTsProdOutMin=[]  UintegralTsProdOutMax=[]  UngainTsProdOutMin=[]  UngainTsProdOutMax=[]  IntegratorContinuousStateAttributes=''  IntegratorStateMustResolveToSignalObject=off  IntegratorRTWStateStorageClass=Auto  FilterContinuousStateAttributes=''  FilterStateMustResolveToSignalObject=off  FilterRTWStateStorageClass=Auto  ParallelPVariant=InternalParameters  IdealPVariant=Disabled  IVariant=InternalParameters  DVariant=Disabled  IntegratorVariant=Continuous  SatVariant=Disabled  AWVariant=Passthrough  PCopyVariant=Disabled  TRVariant=Disabled  FdbkBlocksVariant=Forward  IdealPFdbkVariant=Disabled  SatFdbkVariant=Disabled  DerivativeFilterVariant=Disabled  NVariant=Disabled  NCopyVariant=Disabled_SignalSpec  FilterICVariant=Disabled  IntegratorICVariant=InternalICs  ExternalResetVariant=Disabled  TRSumVariant=Passthrough  SumFdbkVariant=Disabled  SumVariant=Sum_PI  TsampFilterVariant=InternalTs  TsampNgainVariant=Passthrough  TsampIntegralVariant=Passthrough  ExternalSaturationOutDataTypeStr=Inherit: Same as second input  aMode=0
  Discrete model : Scope  Commented=on
  Discrete model1 : Scope
  Echte Ts : Scope  Commented=on
  Echte Ts1 : Scope  Commented=on
  Equal : RelationalOperator  Commented=on  Operator=~=  OutDataTypeStr=boolean  RndMeth=Simplest  InputSameDT=off
  Equal1 : RelationalOperator  Commented=on  Operator===  OutDataTypeStr=boolean  RndMeth=Simplest  InputSameDT=off
  Equal4 : RelationalOperator  Commented=on  Operator=~=  OutDataTypeStr=boolean  RndMeth=Simplest  InputSameDT=off
  Equal5 : RelationalOperator  Commented=on  Operator===  OutDataTypeStr=boolean  RndMeth=Simplest  InputSameDT=off
  Gain : Gain  Commented=on  Gain=17.2
  Gain1 : Gain  Commented=on  Gain=73.4
  Gain2 : Gain  Commented=on  Gain=5
  Gain3 : Gain  Commented=on  Gain=75.2
  Gain5 : Gain  Commented=on  Gain=5
  Hoeveel Tf veraderen : Scope  Commented=on
  Hoeveel Tf veraderen1 : Scope  Commented=on
  Hold U{,1..6} (7 alike) : ZeroOrderHold  Commented=on
  Hold measurement{1..7} (7 alike) : ZeroOrderHold  Commented=on
  Integrator{,1..16} (17 alike) : Integrator  Commented=on
  Ki : Gain  Commented=on  Gain=2.0279e-07
  "Ki " : Gain  Commented=on  Gain=0.00136
  Ki{1..5,13} (6 alike) : Gain  Commented=on  Gain=2.0279e-05
  Ki10 : Gain  Commented=on  Gain=0.0000436
  Ki11 : Gain  Commented=on  Gain=0.00136
  Ki12 : Gain  Commented=on  Gain=0.0000136
  Ki14 : Gain  Commented=on  Gain=0.0000436
  Ki6 : Gain  Commented=on  Gain=0.000136
  Ki7 : Gain  Commented=on  Gain=0.000136
  Ki8 : Gain  Commented=on  Gain=0.000136
  Ki9 : Gain  Commented=on  Gain=0.0000136
  Kp{,1,3..4} (4 alike) : Gain  Commented=on  Gain=7.74
  "Kp " : Gain  Commented=on  Gain=33.84
  Kp10 : Gain  Commented=on  Gain=12
  Kp11 : Gain  Commented=on  Gain=33.84
  Kp12 : Gain  Commented=on  Gain=7
  Kp13 : Gain  Commented=on
  Kp14 : Gain  Commented=on  Gain=12
  Kp2 : Gain  Commented=on
  Kp5 : Gain  Commented=on  Gain=15
  Kp6 : Gain  Commented=on  Gain=12
  Kp7 : Gain  Commented=on  Gain=11
  Kp8 : Gain  Commented=on  Gain=15
  Kp9 : Gain  Commented=on  Gain=7
  Kt{,1..3} (4 alike) : Gain  Commented=on  Gain=0.00045
  "Kt " : Gain  Commented=on  Gain=0.01166
  Kt{4..8,10} (6 alike) : Gain  Commented=on  Gain=0.01166
  Kt9 : Gain  Commented=on  Gain=0.000368
  OL met saturatie : Scope  Commented=on  NumInputPorts=3
  OL met saturatie 2 : Scope  Commented=on  NumInputPorts=3
  OL zonder saturatie{,1..2,4} (4 alike) : Scope  Commented=on
  PID Controller : slpidlib/PID Controller  Commented=on  Controller=PI  Form=Parallel  TimeDomain=Continuous-time  UseExternalTs=off  SampleTime=-1  IntegratorMethod=Forward Euler  FilterMethod=Forward Euler  ControllerParametersSource=internal  P=12  I=0.0000436  UseKiTs=off  D=0  N=100  UseFilter=on  TunerSelectOption=Transfer Function Based (PID Tuner App)  InitialConditionSource=internal  InitialConditionForIntegrator=0  InitialConditionForFilter=0  DifferentiatorICPrevScaledInput=0  ExternalReset=none  TrackingMode=off  Kt=1  LimitOutput=off  SatLimitsSource=internal  UpperSaturationLimit=inf  LowerSaturationLimit=-inf  LinearizeAsGain=on  AntiWindupMode=none  Kb=1  POutMin=[]  POutMax=[]  IOutMin=[]  IOutMax=[]  DOutMin=[]  DOutMax=[]  NOutMin=[]  NOutMax=[]  SumOutMin=[]  SumOutMax=[]  SaturationOutMin=[]  SaturationOutMax=[]  PParamMin=[]  PParamMax=[]  IParamMin=[]  IParamMax=[]  DParamMin=[]  DParamMax=[]  NParamMin=[]  NParamMax=[]  KbParamMin=[]  KbParamMax=[]  KtParamMin=[]  KtParamMax=[]  KbOutMin=[]  KbOutMax=[]  KtOutMin=[]  KtOutMax=[]  IntegratorOutMin=[]  IntegratorOutMax=[]  FilterOutMin=[]  FilterOutMax=[]  SumI1OutMin=[]  SumI1OutMax=[]  SumI2OutMin=[]  SumI2OutMax=[]  SumI3OutMin=[]  SumI3OutMax=[]  SumI4OutMin=[]  SumI4OutMax=[]  SumDOutMin=[]  SumDOutMax=[]  DifferentiatorOutMin=[]  DifferentiatorOutMax=[]  FilterDiffOutCoefMin=[]  FilterDiffOutCoefMax=[]  ReciprocalOutMin=[]  ReciprocalOutMax=[]  SumDenOutMin=[]  SumDenOutMax=[]  SumNumOutMin=[]  SumNumOutMax=[]  DivideOutMin=[]  DivideOutMax=[]  UdiffTsProdOutMin=[]  UdiffTsProdOutMax=[]  NTsProdOutMin=[]  NTsProdOutMax=[]  UintegralTsProdOutMin=[]  UintegralTsProdOutMax=[]  UngainTsProdOutMin=[]  UngainTsProdOutMax=[]  IntegratorContinuousStateAttributes=''  IntegratorStateMustResolveToSignalObject=off  IntegratorRTWStateStorageClass=Auto  FilterContinuousStateAttributes=''  FilterStateMustResolveToSignalObject=off  FilterRTWStateStorageClass=Auto  ParallelPVariant=InternalParameters  IdealPVariant=Disabled  IVariant=InternalParameters  DVariant=Disabled  IntegratorVariant=Continuous  SatVariant=Disabled  AWVariant=Passthrough  PCopyVariant=Disabled  TRVariant=Disabled  FdbkBlocksVariant=Forward  IdealPFdbkVariant=Disabled  SatFdbkVariant=Disabled  DerivativeFilterVariant=Disabled  NVariant=Disabled  NCopyVariant=Disabled_SignalSpec  FilterICVariant=Disabled  IntegratorICVariant=InternalICs  ExternalResetVariant=Disabled  TRSumVariant=Passthrough  SumFdbkVariant=Disabled  SumVariant=Sum_PI  TsampFilterVariant=InternalTs  TsampNgainVariant=Passthrough  TsampIntegralVariant=Passthrough  ExternalSaturationOutDataTypeStr=Inherit: Same as second input  aMode=0
  PID Controller (Gv)1 : slpidlib/PID Controller  Commented=on  Controller=PI  Form=Parallel  TimeDomain=Continuous-time  UseExternalTs=off  SampleTime=-1  IntegratorMethod=Forward Euler  FilterMethod=Forward Euler  ControllerParametersSource=internal  P=1  I=0  UseKiTs=off  D=0  N=100  UseFilter=on  TunerSelectOption=Transfer Function Based (PID Tuner App)  InitialConditionSource=internal  InitialConditionForIntegrator=0  InitialConditionForFilter=0  DifferentiatorICPrevScaledInput=0  ExternalReset=none  TrackingMode=off  Kt=1  LimitOutput=on  SatLimitsSource=internal  UpperSaturationLimit=2  LowerSaturationLimit=-1  LinearizeAsGain=on  AntiWindupMode=clamping  Kb=1  POutMin=[]  POutMax=[]  IOutMin=[]  IOutMax=[]  DOutMin=[]  DOutMax=[]  NOutMin=[]  NOutMax=[]  SumOutMin=[]  SumOutMax=[]  SaturationOutMin=[]  SaturationOutMax=[]  PParamMin=[]  PParamMax=[]  IParamMin=[]  IParamMax=[]  DParamMin=[]  DParamMax=[]  NParamMin=[]  NParamMax=[]  KbParamMin=[]  KbParamMax=[]  KtParamMin=[]  KtParamMax=[]  KbOutMin=[]  KbOutMax=[]  KtOutMin=[]  KtOutMax=[]  IntegratorOutMin=[]  IntegratorOutMax=[]  FilterOutMin=[]  FilterOutMax=[]  SumI1OutMin=[]  SumI1OutMax=[]  SumI2OutMin=[]  SumI2OutMax=[]  SumI3OutMin=[]  SumI3OutMax=[]  SumI4OutMin=[]  SumI4OutMax=[]  SumDOutMin=[]  SumDOutMax=[]  DifferentiatorOutMin=[]  DifferentiatorOutMax=[]  FilterDiffOutCoefMin=[]  FilterDiffOutCoefMax=[]  ReciprocalOutMin=[]  ReciprocalOutMax=[]  SumDenOutMin=[]  SumDenOutMax=[]  SumNumOutMin=[]  SumNumOutMax=[]  DivideOutMin=[]  DivideOutMax=[]  UdiffTsProdOutMin=[]  UdiffTsProdOutMax=[]  NTsProdOutMin=[]  NTsProdOutMax=[]  UintegralTsProdOutMin=[]  UintegralTsProdOutMax=[]  UngainTsProdOutMin=[]  UngainTsProdOutMax=[]  IntegratorContinuousStateAttributes=''  IntegratorStateMustResolveToSignalObject=off  IntegratorRTWStateStorageClass=Auto  FilterContinuousStateAttributes=''  FilterStateMustResolveToSignalObject=off  FilterRTWStateStorageClass=Auto  ParallelPVariant=InternalParameters  IdealPVariant=Disabled  IVariant=InternalParameters  DVariant=Disabled  IntegratorVariant=Continuous  SatVariant=Enabled  AWVariant=ContClampingParallel  PCopyVariant=Disabled  TRVariant=Disabled  FdbkBlocksVariant=Forward  IdealPFdbkVariant=Disabled  SatFdbkVariant=Disabled  DerivativeFilterVariant=Disabled  NVariant=Disabled  NCopyVariant=Disabled_SignalSpec  FilterICVariant=Disabled  IntegratorICVariant=InternalICs  ExternalResetVariant=Disabled  TRSumVariant=Passthrough  SumFdbkVariant=Disabled  SumVariant=Sum_PI  TsampFilterVariant=InternalTs  TsampNgainVariant=Passthrough  TsampIntegralVariant=Passthrough  ExternalSaturationOutDataTypeStr=Inherit: Same as second input  aMode=0
  PID Controller (Gv)2 : slpidlib/PID Controller  Commented=on  Controller=PI  Form=Parallel  TimeDomain=Continuous-time  UseExternalTs=off  SampleTime=-1  IntegratorMethod=Forward Euler  FilterMethod=Forward Euler  ControllerParametersSource=internal  P=1  I=0  UseKiTs=off  D=0  N=100  UseFilter=on  TunerSelectOption=Transfer Function Based (PID Tuner App)  InitialConditionSource=internal  InitialConditionForIntegrator=0  InitialConditionForFilter=0  DifferentiatorICPrevScaledInput=0  ExternalReset=none  TrackingMode=off  Kt=1  LimitOutput=on  SatLimitsSource=internal  UpperSaturationLimit=2  LowerSaturationLimit=-1  LinearizeAsGain=on  AntiWindupMode=clamping  Kb=1  POutMin=[]  POutMax=[]  IOutMin=[]  IOutMax=[]  DOutMin=[]  DOutMax=[]  NOutMin=[]  NOutMax=[]  SumOutMin=[]  SumOutMax=[]  SaturationOutMin=[]  SaturationOutMax=[]  PParamMin=[]  PParamMax=[]  IParamMin=[]  IParamMax=[]  DParamMin=[]  DParamMax=[]  NParamMin=[]  NParamMax=[]  KbParamMin=[]  KbParamMax=[]  KtParamMin=[]  KtParamMax=[]  KbOutMin=[]  KbOutMax=[]  KtOutMin=[]  KtOutMax=[]  IntegratorOutMin=[]  IntegratorOutMax=[]  FilterOutMin=[]  FilterOutMax=[]  SumI1OutMin=[]  SumI1OutMax=[]  SumI2OutMin=[]  SumI2OutMax=[]  SumI3OutMin=[]  SumI3OutMax=[]  SumI4OutMin=[]  SumI4OutMax=[]  SumDOutMin=[]  SumDOutMax=[]  DifferentiatorOutMin=[]  DifferentiatorOutMax=[]  FilterDiffOutCoefMin=[]  FilterDiffOutCoefMax=[]  ReciprocalOutMin=[]  ReciprocalOutMax=[]  SumDenOutMin=[]  SumDenOutMax=[]  SumNumOutMin=[]  SumNumOutMax=[]  DivideOutMin=[]  DivideOutMax=[]  UdiffTsProdOutMin=[]  UdiffTsProdOutMax=[]  NTsProdOutMin=[]  NTsProdOutMax=[]  UintegralTsProdOutMin=[]  UintegralTsProdOutMax=[]  UngainTsProdOutMin=[]  UngainTsProdOutMax=[]  IntegratorContinuousStateAttributes=''  IntegratorStateMustResolveToSignalObject=off  IntegratorRTWStateStorageClass=Auto  FilterContinuousStateAttributes=''  FilterStateMustResolveToSignalObject=off  FilterRTWStateStorageClass=Auto  ParallelPVariant=InternalParameters  IdealPVariant=Disabled  IVariant=InternalParameters  DVariant=Disabled  IntegratorVariant=Continuous  SatVariant=Enabled  AWVariant=ContClampingParallel  PCopyVariant=Disabled  TRVariant=Disabled  FdbkBlocksVariant=Forward  IdealPFdbkVariant=Disabled  SatFdbkVariant=Disabled  DerivativeFilterVariant=Disabled  NVariant=Disabled  NCopyVariant=Disabled_SignalSpec  FilterICVariant=Disabled  IntegratorICVariant=InternalICs  ExternalResetVariant=Disabled  TRSumVariant=Passthrough  SumFdbkVariant=Disabled  SumVariant=Sum_PI  TsampFilterVariant=InternalTs  TsampNgainVariant=Passthrough  TsampIntegralVariant=Passthrough  ExternalSaturationOutDataTypeStr=Inherit: Same as second input  aMode=0
  PID Controller1 : slpidlib/PID Controller  Commented=on  Controller=PI  Form=Parallel  TimeDomain=Continuous-time  UseExternalTs=off  SampleTime=-1  IntegratorMethod=Forward Euler  FilterMethod=Forward Euler  ControllerParametersSource=internal  P=7.74  I=2.0279e-07  UseKiTs=off  D=0  N=100  UseFilter=on  TunerSelectOption=Transfer Function Based (PID Tuner App)  InitialConditionSource=internal  InitialConditionForIntegrator=0  InitialConditionForFilter=0  DifferentiatorICPrevScaledInput=0  ExternalReset=none  TrackingMode=off  Kt=1  LimitOutput=off  SatLimitsSource=internal  UpperSaturationLimit=inf  LowerSaturationLimit=-inf  LinearizeAsGain=on  AntiWindupMode=none  Kb=1  POutMin=[]  POutMax=[]  IOutMin=[]  IOutMax=[]  DOutMin=[]  DOutMax=[]  NOutMin=[]  NOutMax=[]  SumOutMin=[]  SumOutMax=[]  SaturationOutMin=[]  SaturationOutMax=[]  PParamMin=[]  PParamMax=[]  IParamMin=[]  IParamMax=[]  DParamMin=[]  DParamMax=[]  NParamMin=[]  NParamMax=[]  KbParamMin=[]  KbParamMax=[]  KtParamMin=[]  KtParamMax=[]  KbOutMin=[]  KbOutMax=[]  KtOutMin=[]  KtOutMax=[]  IntegratorOutMin=[]  IntegratorOutMax=[]  FilterOutMin=[]  FilterOutMax=[]  SumI1OutMin=[]  SumI1OutMax=[]  SumI2OutMin=[]  SumI2OutMax=[]  SumI3OutMin=[]  SumI3OutMax=[]  SumI4OutMin=[]  SumI4OutMax=[]  SumDOutMin=[]  SumDOutMax=[]  DifferentiatorOutMin=[]  DifferentiatorOutMax=[]  FilterDiffOutCoefMin=[]  FilterDiffOutCoefMax=[]  ReciprocalOutMin=[]  ReciprocalOutMax=[]  SumDenOutMin=[]  SumDenOutMax=[]  SumNumOutMin=[]  SumNumOutMax=[]  DivideOutMin=[]  DivideOutMax=[]  UdiffTsProdOutMin=[]  UdiffTsProdOutMax=[]  NTsProdOutMin=[]  NTsProdOutMax=[]  UintegralTsProdOutMin=[]  UintegralTsProdOutMax=[]  UngainTsProdOutMin=[]  UngainTsProdOutMax=[]  IntegratorContinuousStateAttributes=''  IntegratorStateMustResolveToSignalObject=off  IntegratorRTWStateStorageClass=Auto  FilterContinuousStateAttributes=''  FilterStateMustResolveToSignalObject=off  FilterRTWStateStorageClass=Auto  ParallelPVariant=InternalParameters  IdealPVariant=Disabled  IVariant=InternalParameters  DVariant=Disabled  IntegratorVariant=Continuous  SatVariant=Disabled  AWVariant=Passthrough  PCopyVariant=Disabled  TRVariant=Disabled  FdbkBlocksVariant=Forward  IdealPFdbkVariant=Disabled  SatFdbkVariant=Disabled  DerivativeFilterVariant=Disabled  NVariant=Disabled  NCopyVariant=Disabled_SignalSpec  FilterICVariant=Disabled  IntegratorICVariant=InternalICs  ExternalResetVariant=Disabled  TRSumVariant=Passthrough  SumFdbkVariant=Disabled  SumVariant=Sum_PI  TsampFilterVariant=InternalTs  TsampNgainVariant=Passthrough  TsampIntegralVariant=Passthrough  ExternalSaturationOutDataTypeStr=Inherit: Same as second input  aMode=0
  PID Controller2 : slpidlib/PID Controller  Commented=on  Controller=PI  Form=Parallel  TimeDomain=Continuous-time  UseExternalTs=off  SampleTime=-1  IntegratorMethod=Forward Euler  FilterMethod=Forward Euler  ControllerParametersSource=internal  P=7.74  I=0  UseKiTs=off  D=0  N=100  UseFilter=on  TunerSelectOption=Transfer Function Based (PID Tuner App)  InitialConditionSource=internal  InitialConditionForIntegrator=0  InitialConditionForFilter=0  DifferentiatorICPrevScaledInput=0  ExternalReset=none  TrackingMode=off  Kt=1  LimitOutput=off  SatLimitsSource=internal  UpperSaturationLimit=inf  LowerSaturationLimit=-inf  LinearizeAsGain=on  AntiWindupMode=none  Kb=1  POutMin=[]  POutMax=[]  IOutMin=[]  IOutMax=[]  DOutMin=[]  DOutMax=[]  NOutMin=[]  NOutMax=[]  SumOutMin=[]  SumOutMax=[]  SaturationOutMin=[]  SaturationOutMax=[]  PParamMin=[]  PParamMax=[]  IParamMin=[]  IParamMax=[]  DParamMin=[]  DParamMax=[]  NParamMin=[]  NParamMax=[]  KbParamMin=[]  KbParamMax=[]  KtParamMin=[]  KtParamMax=[]  KbOutMin=[]  KbOutMax=[]  KtOutMin=[]  KtOutMax=[]  IntegratorOutMin=[]  IntegratorOutMax=[]  FilterOutMin=[]  FilterOutMax=[]  SumI1OutMin=[]  SumI1OutMax=[]  SumI2OutMin=[]  SumI2OutMax=[]  SumI3OutMin=[]  SumI3OutMax=[]  SumI4OutMin=[]  SumI4OutMax=[]  SumDOutMin=[]  SumDOutMax=[]  DifferentiatorOutMin=[]  DifferentiatorOutMax=[]  FilterDiffOutCoefMin=[]  FilterDiffOutCoefMax=[]  ReciprocalOutMin=[]  ReciprocalOutMax=[]  SumDenOutMin=[]  SumDenOutMax=[]  SumNumOutMin=[]  SumNumOutMax=[]  DivideOutMin=[]  DivideOutMax=[]  UdiffTsProdOutMin=[]  UdiffTsProdOutMax=[]  NTsProdOutMin=[]  NTsProdOutMax=[]  UintegralTsProdOutMin=[]  UintegralTsProdOutMax=[]  UngainTsProdOutMin=[]  UngainTsProdOutMax=[]  IntegratorContinuousStateAttributes=''  IntegratorStateMustResolveToSignalObject=off  IntegratorRTWStateStorageClass=Auto  FilterContinuousStateAttributes=''  FilterStateMustResolveToSignalObject=off  FilterRTWStateStorageClass=Auto  ParallelPVariant=InternalParameters  IdealPVariant=Disabled  IVariant=InternalParameters  DVariant=Disabled  IntegratorVariant=Continuous  SatVariant=Disabled  AWVariant=Passthrough  PCopyVariant=Disabled  TRVariant=Disabled  FdbkBlocksVariant=Forward  IdealPFdbkVariant=Disabled  SatFdbkVariant=Disabled  DerivativeFilterVariant=Disabled  NVariant=Disabled  NCopyVariant=Disabled_SignalSpec  FilterICVariant=Disabled  IntegratorICVariant=InternalICs  ExternalResetVariant=Disabled  TRSumVariant=Passthrough  SumFdbkVariant=Disabled  SumVariant=Sum_PI  TsampFilterVariant=InternalTs  TsampNgainVariant=Passthrough  TsampIntegralVariant=Passthrough  ExternalSaturationOutDataTypeStr=Inherit: Same as second input  aMode=0
  PID Controller4 : slpidlib/PID Controller  Commented=on  Controller=PI  Form=Parallel  TimeDomain=Continuous-time  UseExternalTs=off  SampleTime=-1  IntegratorMethod=Forward Euler  FilterMethod=Forward Euler  ControllerParametersSource=internal  P=7.74  I=0  UseKiTs=off  D=0  N=100  UseFilter=on  TunerSelectOption=Transfer Function Based (PID Tuner App)  InitialConditionSource=internal  InitialConditionForIntegrator=0  InitialConditionForFilter=0  DifferentiatorICPrevScaledInput=0  ExternalReset=none  TrackingMode=off  Kt=1  LimitOutput=off  SatLimitsSource=internal  UpperSaturationLimit=inf  LowerSaturationLimit=-inf  LinearizeAsGain=on  AntiWindupMode=none  Kb=1  POutMin=[]  POutMax=[]  IOutMin=[]  IOutMax=[]  DOutMin=[]  DOutMax=[]  NOutMin=[]  NOutMax=[]  SumOutMin=[]  SumOutMax=[]  SaturationOutMin=[]  SaturationOutMax=[]  PParamMin=[]  PParamMax=[]  IParamMin=[]  IParamMax=[]  DParamMin=[]  DParamMax=[]  NParamMin=[]  NParamMax=[]  KbParamMin=[]  KbParamMax=[]  KtParamMin=[]  KtParamMax=[]  KbOutMin=[]  KbOutMax=[]  KtOutMin=[]  KtOutMax=[]  IntegratorOutMin=[]  IntegratorOutMax=[]  FilterOutMin=[]  FilterOutMax=[]  SumI1OutMin=[]  SumI1OutMax=[]  SumI2OutMin=[]  SumI2OutMax=[]  SumI3OutMin=[]  SumI3OutMax=[]  SumI4OutMin=[]  SumI4OutMax=[]  SumDOutMin=[]  SumDOutMax=[]  DifferentiatorOutMin=[]  DifferentiatorOutMax=[]  FilterDiffOutCoefMin=[]  FilterDiffOutCoefMax=[]  ReciprocalOutMin=[]  ReciprocalOutMax=[]  SumDenOutMin=[]  SumDenOutMax=[]  SumNumOutMin=[]  SumNumOutMax=[]  DivideOutMin=[]  DivideOutMax=[]  UdiffTsProdOutMin=[]  UdiffTsProdOutMax=[]  NTsProdOutMin=[]  NTsProdOutMax=[]  UintegralTsProdOutMin=[]  UintegralTsProdOutMax=[]  UngainTsProdOutMin=[]  UngainTsProdOutMax=[]  IntegratorContinuousStateAttributes=''  IntegratorStateMustResolveToSignalObject=off  IntegratorRTWStateStorageClass=Auto  FilterContinuousStateAttributes=''  FilterStateMustResolveToSignalObject=off  FilterRTWStateStorageClass=Auto  ParallelPVariant=InternalParameters  IdealPVariant=Disabled  IVariant=InternalParameters  DVariant=Disabled  IntegratorVariant=Continuous  SatVariant=Disabled  AWVariant=Passthrough  PCopyVariant=Disabled  TRVariant=Disabled  FdbkBlocksVariant=Forward  IdealPFdbkVariant=Disabled  SatFdbkVariant=Disabled  DerivativeFilterVariant=Disabled  NVariant=Disabled  NCopyVariant=Disabled_SignalSpec  FilterICVariant=Disabled  IntegratorICVariant=InternalICs  ExternalResetVariant=Disabled  TRSumVariant=Passthrough  SumFdbkVariant=Disabled  SumVariant=Sum_PI  TsampFilterVariant=InternalTs  TsampNgainVariant=Passthrough  TsampIntegralVariant=Passthrough  ExternalSaturationOutDataTypeStr=Inherit: Same as second input  aMode=0
  PID Controller6 : slpidlib/PID Controller  Commented=on  Controller=PI  Form=Parallel  TimeDomain=Continuous-time  UseExternalTs=off  SampleTime=-1  IntegratorMethod=Forward Euler  FilterMethod=Forward Euler  ControllerParametersSource=internal  P=7.74  I=0  UseKiTs=off  D=0  N=100  UseFilter=on  TunerSelectOption=Transfer Function Based (PID Tuner App)  InitialConditionSource=internal  InitialConditionForIntegrator=0  InitialConditionForFilter=0  DifferentiatorICPrevScaledInput=0  ExternalReset=none  TrackingMode=off  Kt=1  LimitOutput=off  SatLimitsSource=internal  UpperSaturationLimit=inf  LowerSaturationLimit=-inf  LinearizeAsGain=on  AntiWindupMode=none  Kb=1  POutMin=[]  POutMax=[]  IOutMin=[]  IOutMax=[]  DOutMin=[]  DOutMax=[]  NOutMin=[]  NOutMax=[]  SumOutMin=[]  SumOutMax=[]  SaturationOutMin=[]  SaturationOutMax=[]  PParamMin=[]  PParamMax=[]  IParamMin=[]  IParamMax=[]  DParamMin=[]  DParamMax=[]  NParamMin=[]  NParamMax=[]  KbParamMin=[]  KbParamMax=[]  KtParamMin=[]  KtParamMax=[]  KbOutMin=[]  KbOutMax=[]  KtOutMin=[]  KtOutMax=[]  IntegratorOutMin=[]  IntegratorOutMax=[]  FilterOutMin=[]  FilterOutMax=[]  SumI1OutMin=[]  SumI1OutMax=[]  SumI2OutMin=[]  SumI2OutMax=[]  SumI3OutMin=[]  SumI3OutMax=[]  SumI4OutMin=[]  SumI4OutMax=[]  SumDOutMin=[]  SumDOutMax=[]  DifferentiatorOutMin=[]  DifferentiatorOutMax=[]  FilterDiffOutCoefMin=[]  FilterDiffOutCoefMax=[]  ReciprocalOutMin=[]  ReciprocalOutMax=[]  SumDenOutMin=[]  SumDenOutMax=[]  SumNumOutMin=[]  SumNumOutMax=[]  DivideOutMin=[]  DivideOutMax=[]  UdiffTsProdOutMin=[]  UdiffTsProdOutMax=[]  NTsProdOutMin=[]  NTsProdOutMax=[]  UintegralTsProdOutMin=[]  UintegralTsProdOutMax=[]  UngainTsProdOutMin=[]  UngainTsProdOutMax=[]  IntegratorContinuousStateAttributes=''  IntegratorStateMustResolveToSignalObject=off  IntegratorRTWStateStorageClass=Auto  FilterContinuousStateAttributes=''  FilterStateMustResolveToSignalObject=off  FilterRTWStateStorageClass=Auto  ParallelPVariant=InternalParameters  IdealPVariant=Disabled  IVariant=InternalParameters  DVariant=Disabled  IntegratorVariant=Continuous  SatVariant=Disabled  AWVariant=Passthrough  PCopyVariant=Disabled  TRVariant=Disabled  FdbkBlocksVariant=Forward  IdealPFdbkVariant=Disabled  SatFdbkVariant=Disabled  DerivativeFilterVariant=Disabled  NVariant=Disabled  NCopyVariant=Disabled_SignalSpec  FilterICVariant=Disabled  IntegratorICVariant=InternalICs  ExternalResetVariant=Disabled  TRSumVariant=Passthrough  SumFdbkVariant=Disabled  SumVariant=Sum_PI  TsampFilterVariant=InternalTs  TsampNgainVariant=Passthrough  TsampIntegralVariant=Passthrough  ExternalSaturationOutDataTypeStr=Inherit: Same as second input  aMode=0
  PID Controller7 : slpidlib/PID Controller  Commented=on  Controller=PI  Form=Parallel  TimeDomain=Discrete-time  UseExternalTs=off  SampleTime=-1  IntegratorMethod=Forward Euler  FilterMethod=Forward Euler  ControllerParametersSource=internal  P=1  I=1  UseKiTs=off  D=0  N=100  UseFilter=on  TunerSelectOption=Transfer Function Based (PID Tuner App)  InitialConditionSource=internal  InitialConditionForIntegrator=0  InitialConditionForFilter=0  DifferentiatorICPrevScaledInput=0  ExternalReset=none  TrackingMode=off  Kt=1  LimitOutput=off  SatLimitsSource=internal  UpperSaturationLimit=inf  LowerSaturationLimit=-inf  LinearizeAsGain=on  AntiWindupMode=none  Kb=1  POutMin=[]  POutMax=[]  IOutMin=[]  IOutMax=[]  DOutMin=[]  DOutMax=[]  NOutMin=[]  NOutMax=[]  SumOutMin=[]  SumOutMax=[]  SaturationOutMin=[]  SaturationOutMax=[]  PParamMin=[]  PParamMax=[]  IParamMin=[]  IParamMax=[]  DParamMin=[]  DParamMax=[]  NParamMin=[]  NParamMax=[]  KbParamMin=[]  KbParamMax=[]  KtParamMin=[]  KtParamMax=[]  KbOutMin=[]  KbOutMax=[]  KtOutMin=[]  KtOutMax=[]  IntegratorOutMin=[]  IntegratorOutMax=[]  FilterOutMin=[]  FilterOutMax=[]  SumI1OutMin=[]  SumI1OutMax=[]  SumI2OutMin=[]  SumI2OutMax=[]  SumI3OutMin=[]  SumI3OutMax=[]  SumI4OutMin=[]  SumI4OutMax=[]  SumDOutMin=[]  SumDOutMax=[]  DifferentiatorOutMin=[]  DifferentiatorOutMax=[]  FilterDiffOutCoefMin=[]  FilterDiffOutCoefMax=[]  ReciprocalOutMin=[]  ReciprocalOutMax=[]  SumDenOutMin=[]  SumDenOutMax=[]  SumNumOutMin=[]  SumNumOutMax=[]  DivideOutMin=[]  DivideOutMax=[]  UdiffTsProdOutMin=[]  UdiffTsProdOutMax=[]  NTsProdOutMin=[]  NTsProdOutMax=[]  UintegralTsProdOutMin=[]  UintegralTsProdOutMax=[]  UngainTsProdOutMin=[]  UngainTsProdOutMax=[]  IntegratorContinuousStateAttributes=''  IntegratorStateMustResolveToSignalObject=off  IntegratorRTWStateStorageClass=Auto  FilterContinuousStateAttributes=''  FilterStateMustResolveToSignalObject=off  FilterRTWStateStorageClass=Auto  ParallelPVariant=InternalParameters  IdealPVariant=Disabled  IVariant=InternalParameters  DVariant=Disabled  IntegratorVariant=Discrete  SatVariant=Disabled  AWVariant=Passthrough  PCopyVariant=Disabled  TRVariant=Disabled  FdbkBlocksVariant=Forward  IdealPFdbkVariant=Disabled  SatFdbkVariant=Disabled  DerivativeFilterVariant=Disabled  NVariant=Disabled  NCopyVariant=Disabled_SignalSpec  FilterICVariant=Disabled  IntegratorICVariant=InternalICs  ExternalResetVariant=Disabled  TRSumVariant=Passthrough  SumFdbkVariant=Disabled  SumVariant=Sum_PI  TsampFilterVariant=InternalTs  TsampNgainVariant=Passthrough  TsampIntegralVariant=Passthrough  ExternalSaturationOutDataTypeStr=Inherit: Same as second input  aMode=0
  "Plant " : cstblocks/LTI System  Commented=on  sys=tf(numAdjdelay,denAdjdelay)  IC=[]
  Plant H1 : cstblocks/LTI System  Commented=on  sys=tf(numAdjZdelay,denAdjZdelay)  IC=[]
  Plant H{2..12,14..17,19,21..23,25..26} (21 alike) : cstblocks/LTI System  Commented=on  sys=tf(numAdjdelay,denAdjdelay)  IC=[]
  Plant H13 : cstblocks/LTI System  Commented=on  sys=tf(numAdjZdelay,denAdjZdelay)  IC=[]
  Plant continious : cstblocks/LTI System  Commented=on  sys=tf(numAdjdelay,denAdjdelay)  IC=[]
  Plant discrete : cstblocks/LTI System  Commented=on  sys=tf(numAdjdelay,denAdjdelay)  IC=[]
  Plant discrete1 : cstblocks/LTI System  Commented=on  sys=tf(numAdjdelay,denAdjdelay)  IC=[]
  Plant discrete2 : cstblocks/LTI System  sys=tf(numAdjdelay,denAdjdelay)  IC=[]
  Plant discrete3 : cstblocks/LTI System  sys=tf(numAdjdelay,denAdjdelay)  IC=[]
  Plant discrete4 : cstblocks/LTI System  sys=tf(numAdjdelay,denAdjdelay)  IC=[]
  Rate Limiter{,1..9} (10 alike) : RateLimiter  Commented=on  RisingSlewLimit=0.000006  FallingSlewLimit=-0.0000238  SampleTimeMode=inherited
  Saturation{1..23} (23 alike) : Saturate  Commented=on  UpperLimit=2  LowerLimit=-1
  Saturation24 : Saturate  UpperLimit=2  LowerLimit=-1
  Scope{,5,10,13,20,23} (6 alike) : Scope  Commented=on  NumInputPorts=2
  Scope{1..3,12,16,19} (6 alike) : Scope  Commented=on  NumInputPorts=3
  Scope{4,6..9,11,14..15,17..18,25..29,31..34} (19 alike) : Scope  Commented=on
  Scope{21..22,24,30,35..36} (6 alike) : Scope
  Scope37 : Scope  NumInputPorts=2
  Scope38 : Scope  NumInputPorts=2
  Sign{,1,4..5} (4 alike) : Signum  Commented=on
  Sine Wave : Sin  Commented=on  SampleTime=0
  Sine Wave1 : Sin  Commented=on  SampleTime=0
  Step : Step  After=-0.1  SampleTime=0
  Step -0.0247 : Step  After=-0.0247  SampleTime=0
  Step -2 : Step  After=-1  SampleTime=0
  Step1 : Step  Commented=on  After=-0.25  SampleTime=0  ZeroCross=off
  Step10 : Step  Commented=on  After=-1  SampleTime=0  ZeroCross=off
  Step{2..5,7,9,11,13,16,20} (10 alike) : Step  Commented=on  SampleTime=0
  Step{6,12,15,17,19} (5 alike) : Step  Commented=on  SampleTime=0  ZeroCross=off
  Step8 : Step  Commented=on  After=-1  SampleTime=0  ZeroCross=off
  Sum{,6,17,21,23,27,35,39,41,44,51,55,62,66,70,74,79,84,91,95} (20 alike) : Sum  Commented=on  Inputs=|++  OutDataTypeStr=Inherit: Keep MSB
  Sum{1,3..4,7,9,20,26,30,33..34,36,48,54,58..59,63,65,67,69,73,78,82,87..90,92,94,97,101} (30 alike) : Sum  Commented=on  Inputs=|++
  Sum{2,5,8,10..16,18,22,24,28,31,37..38,40,42..43,45,47,49,52,56,60..61,68,71,75..76,80,83,85,98..99,102} (37 alike) : Sum  Commented=on  Inputs=|+-
  Sum{19,25,29,32,46,50,53,57,64,72,77,81,86,96,100} (15 alike) : Sum  Commented=on  Inputs=+-|
  Sum{103,105,108..111} (6 alike) : Sum  Inputs=|++
  Sum104 : Sum  Inputs=|+-
  Sum106 : Sum  Inputs=|++  OutDataTypeStr=Inherit: Keep MSB
  Sum107 : Sum  Inputs=|+-
  Sum93 : Sum  Inputs=+-|
  Switch : Switch  Commented=on  Criteria=u2 > Threshold  SaturateOnIntegerOverflow=off  InputSameDT=off
  Switch2 : Switch  Commented=on  Criteria=u2 > Threshold  SaturateOnIntegerOverflow=off  InputSameDT=off
  "T Fruit Ref     " : Constant  Commented=on  Value=-1
  T Fruit Ref1 : Constant  Value=-1
  T Fruit Ref2 : Constant  Commented=on  Value=-1
  "T Fruit Zero " : Constant  Commented=on  Value=-0.75
  "T Fruit Zero     " : Constant  Commented=on  Value=-0.75
  T Fruit Zero  1 : Constant  Value=-0.75
  T Fruit Zero  2 : Constant  Commented=on  Value=-0.75
  T Fruit Zero 1 : Constant  Commented=on  Value=-0.75
  T Fruit Zero 2 : Constant  Value=-0.75
  T Fruit Zero 3 : Constant  Value=-0.75
  T Fruit Zero 4 : Constant  Value=-0.75
  "T Set   " : Scope  Commented=on
  T Set   1 : Scope  Commented=on
  T Set   2 : Scope  Commented=on
  T Set   3 : Scope
  T Set   4 : Scope
  T Set   5 : Scope
  T Set Zero {,1..3} (4 alike) : Constant  Commented=on  Value=-1
  T Set Zero 4 : Constant  Value=-1
  T Set Zero 5 : Constant  Value=-1
  T Set Zero 6 : Constant  Value=-1
  "Tfruit   " : Scope  Commented=on
  Tfruit   1 : Scope
  Tfruit   2 : Scope
  Tfruit   3 : Scope
  Tfruit Ref : Constant  Commented=on
  Tfruit dat ge wilt{,1..3} (4 alike) : Constant  Commented=on  Value=-1
  Tfruit real : Scope  Commented=on
  Tfruit real1 : Scope  Commented=on
  Tfruit real2 : Scope  Commented=on
  Tfruit{0,2..3,5} (4 alike) : Constant  Commented=on  Value=-0.75
  Tfruit0'{,1..3} (4 alike) : Constant  Commented=on  Value=-0.75
  Tfruit1 : Scope  Commented=on
  Tfruit4 : Scope  Commented=on
  TfruitRef : Constant  Commented=on  Value=-1
  Tfruitzero : Constant  Commented=on  Value=-0.75
  Time delay : TransportDelay  Commented=on  DelayTime=7860
  Transfer Fcn : TransferFcn  Commented=on  Denominator=[1 1]
  Transport Delay{,1..7,9..12,14,18} (14 alike) : TransportDelay  Commented=on  DelayTime=7806
  Transport Delay{13,15..17,19..24} (10 alike) : TransportDelay  Commented=on  DelayTime=7860
  Transport Delay25 : TransportDelay  Commented=on  DelayTime=7806  BufferSize=26245512
  Transport Delay26 : TransportDelay  DelayTime=7860
  Transport Delay27 : TransportDelay  DelayTime=7860
  Transport Delay28 : TransportDelay  DelayTime=7860
  Transport Delay8 : TransportDelay  Commented=on  DelayTime=7806  BufferSize=26245512
  Ts naar koelcel{,1..3} (4 alike) : Scope  Commented=on
  Tset{0..3} (4 alike) : Constant  Commented=on  Value=-1
  TsetOut : Scope  Commented=on
  TsetZero : Constant  Commented=on  Value=-1
  Zero-Order Hold : ZeroOrderHold  Commented=on  SampleTime=0.01
  Zero-Order Hold1 : ZeroOrderHold  Commented=on  SampleTime=0.01
  Zero-Order Hold10 : ZeroOrderHold  SampleTime=172800
  Zero-Order Hold11 : ZeroOrderHold  SampleTime=172800
  Zero-Order Hold{2..9} (8 alike) : ZeroOrderHold  Commented=on
  delta T discreet{,1..3} (4 alike) : Scope  Commented=on
  Output continious : Outport
  Tfruit : Outport  Port=2
  T Set : Outport  Port=3
  Output : Outport  Port=4
  Output discrete : Outport  Port=5
  wires:
  Plant H1/1 -> Sum9/1, Hoeveel Tf veraderen/1, Sum10/2  "deltaT"
  Sum9/1 -> Tfruit1/1
  Constant4/1 -> Sum9/2
  Sum10/1 -> PID Controller (Gv)1/1  "Error"
  Sum8/1 -> Sum10/1  "R'"
  PID Controller (Gv)1/1 -> Rate Limiter/1  "Delta S"
  Bias1/1 -> Sum7/1
  Sum7/1 -> Echte Ts/1  "DeltaS"
  Constant2/1 -> Sum8/2
  Constant6/1 -> Sum8/1
  Rate Limiter/1 -> Delta S/1, Sum7/2, Transport Delay/1
  Transport Delay/1 -> Plant H1/1
  Transport Delay1/1 -> OL met saturatie/2, Plant H2/1  "U"
  Saturation1/1 -> Scope3/2, Rate Limiter1/1  "Na absolute sat"
  Rate Limiter1/1 -> Scope3/3, Transport Delay1/1  "Na saturatie"
  Step2/1 -> Sum11/1
  Sum11/1 -> OL met saturatie/3, Gain/1  "error"
  Plant H2/1 -> OL met saturatie/1, Sum11/2  "deltaT"
  Gain/1 -> Scope3/1, Saturation1/1  "Voor saturatie"
  Gain1/1 -> Transport Delay2/1
  Transport Delay2/1 -> Plant H3/1
  Step3/1 -> Sum12/1
  Sum12/1 -> Gain1/1
  Plant H3/1 -> OL zonder saturatie/1, Sum12/2
  Step5/1 -> Sum14/1
  Saturation2/1 -> Scope2/2, Rate Limiter2/1  "Na absolute sat"
  Rate Limiter2/1 -> Scope2/3, Transport Delay3/1  "Na saturatie"
  Transport Delay4/1 -> Plant H5/1
  Sum13/1 -> OL met saturatie 2/3, PID Controller1/1  "error"
  Step4/1 -> Sum13/1
  PID Controller1/1 -> Scope2/1, Saturation2/1  "Voor saturatie"
  Plant H5/1 -> OL zonder saturatie2/1, Sum14/2
  Transport Delay3/1 -> OL met saturatie 2/2, Plant H4/1  "U"
  Plant H4/1 -> Scope4/1, OL met saturatie 2/1, Sum13/2  "deltaT"
  Sum14/1 -> PID Controller2/1
  PID Controller2/1 -> Transport Delay4/1  "Voor saturatie"
  PID Controller4/1 -> Transport Delay6/1  "Voor saturatie"
  Sum16/1 -> PID Controller4/1
  Sum/1 -> Anti windup video totale command/3, Saturation3/1  "Voor saturatie"
  Plant H6/1 -> Scope6/1, Sum15/2  "deltaT"
  Plant H7/1 -> OL zonder saturatie1/1, Sum16/2
  Step6/1 -> Sum15/1
  Transport Delay6/1 -> Plant H7/1
  Transport Delay5/1 -> Anti windup video 2 I actie/3, Plant H6/1  "U"
  Saturation3/1 -> Rate Limiter3/1  "Na absolute sat"
  Step7/1 -> Sum16/1
  Rate Limiter3/1 -> Anti windup video totale command/2, Transport Delay5/1  "Na sauratie"
  Ki/1 -> Integrator/1
  Sum15/1 -> Anti windup video 2 I actie/2, Anti windup video totale command/1, Kp/1, Ki/1  "error"
  Integrator/1 -> Anti windup video 2 I actie/1, Sum/1  "I actie"
  Kp/1 -> Sum/2
  Transport Delay7/1 -> Anti windup video 2 I actie1/3, Plant H8/1  "U"
  Sum18/1 -> Anti windup video 2 I actie1/2, Anti windup video totale command1/1, Ki1/1, Kp1/1  "error"
  Rate Limiter4/1 -> Anti windup video totale command1/2, Sum19/1, Transport Delay7/1  "Na sauratie"
  Sum17/1 -> Anti windup video totale command1/3, Sum19/2, Saturation4/1  "Voor saturatie"
  Step8/1 -> Sum18/1
  Plant H8/1 -> Continious model/1, Sum18/2  "deltaT"
  Saturation4/1 -> Rate Limiter4/1  "Na absolute sat"
  Integrator1/1 -> Sum17/2, Anti windup video 2 I actie1/1  "I actie"
  Kp1/1 -> Sum17/1  "P actie"
  Sum19/1 -> Kt/1
  Ki1/1 -> Sum20/1
  Sum20/1 -> Integrator1/1
  Kt/1 -> Sum20/2
  Rate Limiter5/1 -> Anti windup video totale command2/2, Equal/2, Transport Delay8/1  "Na sauratie"
  Saturation5/1 -> Rate Limiter5/1  "Na absolute sat"
  Plant H9/1 -> Scope7/1, Sum22/2  "deltaT"
  Step9/1 -> Sum22/1
  Integrator2/1 -> Sum21/2, Anti windup video 2 I actie clamp/1  "I actie"
  Kp2/1 -> Sum21/1  "P actie"
  Sum22/1 -> Anti windup video 2 I actie clamp/2, Sign/1, Ki2/1, Kp2/1, Anti windup video totale command2/1  "error"
  Sum21/1 -> Anti windup video totale command2/3, Sign1/1, Equal/1, Saturation5/1  "Voor saturatie"
  Transport Delay8/1 -> Anti windup video 2 I actie clamp/3, Plant H9/1  "U"
  Equal1/1 -> AND/1
  Equal/1 -> AND/2
  Switch/1 -> Integrator2/1
  AND/1 -> Switch/2
  Ki2/1 -> Switch/3
  Constant5/1 -> Switch/1
  Sign/1 -> Equal1/1
  Sign1/1 -> Equal1/2
  Sum26/1 -> Integrator3/1
  Plant H10/1 -> Hold measurement1/1  "deltaT"
  Kt1/1 -> Sum26/2
  Sum23/1 -> Anti windup video totale command3/3, Sum25/2, Saturation6/1  "Voor saturatie"
  Sum24/1 -> Anti windup video 2 I actie2/2, Anti windup video totale command3/1, Ki3/1, Kp3/1  "error"
  Integrator3/1 -> Sum23/2, Anti windup video 2 I actie2/1  "I actie"
  Ki3/1 -> Sum26/1
  Saturation6/1 -> Rate Limiter6/1  "Na absolute sat"
  Sum25/1 -> Kt1/1
  Rate Limiter6/1 -> Anti windup video totale command3/2, Sum25/1, Transport Delay9/1  "Na sauratie"
  Step10/1 -> Sum24/1
  Kp3/1 -> Sum23/1  "P actie"
  Transport Delay9/1 -> Anti windup video 2 I actie2/3, Hold U/1  "U"
  Hold U/1 -> Plant H10/1
  Sine Wave/1 -> Gain2/1
  Gain2/1 -> Scope5/2, Zero-Order Hold/1  "Pure"
  Zero-Order Hold/1 -> Scope5/1  "discrete"
  Ki4/1 -> Sum30/1
  Integrator4/1 -> Sum27/2  "I actie"
  Saturation7/1 -> Rate Limiter7/1  "Na absolute sat"
  Rate Limiter7/1 -> Sum3/2, Sum29/1, Transport Delay10/1  "Na sauratie"
  Sum29/1 -> Kt2/1
  Kp4/1 -> Sum27/1  "P actie"
  Sum28/1 -> Ki4/1, Kp4/1  "error"
  Transport Delay10/1 -> Hold U1/1  "U"
  Hold U1/1 -> Plant H11/1
  Plant H11/1 -> Hold measurement3/1  "deltaT"
  Sum30/1 -> Integrator4/1
  Kt2/1 -> Sum30/2
  Sum27/1 -> Saturation7/1, Sum29/2  "Voor saturatie"
  Tfruit0'/1 -> Sum1/2
  Sum2/1 -> Sum28/1
  Tfruit0/1 -> Sum2/2
  Tfruit dat ge wilt/1 -> Sum2/1
  Tset0/1 -> Sum3/1
  Sum3/1 -> Ts naar koelcel/1
  Sum1/1 -> Tfruit real/1
  Tfruit dat ge wilt1/1 -> Sum5/1
  Tfruit0'1/1 -> Sum4/2
  Sum5/1 -> Sum31/1
  Kt3/1 -> Sum34/2
  Sum34/1 -> Integrator5/1
  Plant H12/1 -> Hold U3/1  "deltaT"
  Rate Limiter8/1 -> Sum33/2, Sum32/1, Transport Delay11/1  "Na sauratie"
  Sum32/1 -> Kt3/1
  Kp5/1 -> Sum6/1  "P actie"
  Integrator5/1 -> Sum6/2  "I actie"
  Ki5/1 -> Sum34/1
  Sum6/1 -> Saturation8/1, Sum32/2  "Voor saturatie"
  Saturation8/1 -> Rate Limiter8/1  "Na absolute sat"
  Tfruit2/1 -> Sum5/2
  Sum33/1 -> Ts naar koelcel1/1
  Tset1/1 -> Sum33/1
  Transport Delay11/1 -> Hold U2/1  "U"
  Hold U2/1 -> Plant H12/1
  Sum31/1 -> Ki5/1, Kp5/1  "error"
  Sum4/1 -> Tfruit real1/1
  Hold measurement3/1 -> Sum28/2, Sum1/1, delta T discreet/1
  Hold measurement1/1 -> Sum24/2, Discrete model/1
  Hold U3/1 -> delta T discreet1/1, Sum31/2, Sum4/1  "delta Tf disc"
  Constant1/1 -> Sum68/2
  Hold measurement4/1 -> Sum56/2, Sum36/1, delta T discreet2/1
  Step13/1 -> Sum40/1
  Sum69/1 -> Tfruit4/1
  Sum44/1 -> Anti windup video totale command5/3, Sum46/2, Saturation12/1  "Voor saturatie"
  Plant H22/1 -> OL zonder saturatie4/1, Sum43/2
  Sum68/1 -> Sum37/1  "R'"
  Step16/1 -> Sum43/1
  Zero-Order Hold1/1 -> Scope10/1  "discrete"
  Transport Delay17/1 -> Plant H19/1
  Sum36/1 -> Tfruit real2/1
  Saturation15/1 -> Transport Delay14/1, Sum57/1, Sum58/2  "Na sauratie"
  Kt6/1 -> Sum59/2
  Sum56/1 -> Ki10/1, Kp10/1  "error"
  Sum47/1 -> Sum56/1
  Transport Delay23/1 -> Hold U4/1, Anti windup video 2 I actie5/3  "U"
  Sum67/1 -> Echte Ts1/1  "DeltaS"
  Tfruit3/1 -> Sum47/2
  Sum58/1 -> Ts naar koelcel2/1
  Integrator6/1 -> Anti windup video 2 I actie3/1, Sum35/1, Scope13/1  "I actie"
  Kt4/1 -> Sum48/2
  Sum55/1 -> Saturation15/1, Sum57/2  "Voor saturatie"
  Sum57/1 -> Hold measurement5/1
  Saturation14/1 -> Transport Delay23/1, Sum53/1, Anti windup video totale command7/2  "Na absolute sat"
  Tfruit dat ge wilt2/1 -> Sum47/1
  Ki10/1 -> Sum59/1
  Plant H15/1 -> Hold measurement4/1  "deltaT"
  Integrator10/1 -> Sum55/2  "I actie"
  Gain5/1 -> Scope10/2, Zero-Order Hold1/1  "Pure"
  Ki9/1 -> Sum54/1
  Sum52/1 -> Anti windup video 2 I actie5/2, Anti windup video totale command7/1, Ki9/1, Kp9/1  "error"
  Integrator9/1 -> Sum51/2, Anti windup video 2 I actie5/1  "I actie"
  Ki6/1 -> Integrator6/1
  Kt5/1 -> Sum54/2
  Sine Wave1/1 -> Gain5/1
  Sum46/1 -> Kt4/1
  Saturation9/1 -> Scope/2, Transport Delay13/1  "dTset after saturation"
  Plant H14/1 -> Hold measurement2/1  "deltaT"
  Sum38/1 -> Gain3/1  "error"
  Sum35/1 -> Anti windup video totale command4/3, Saturation11/1  "Voor saturatie"
  Tset2/1 -> Sum58/1
  Sum43/1 -> PID Controller6/1
  Kp7/1 -> Sum44/1  "P actie"
  Bias2/1 -> Sum67/1
  Integrator7/1 -> Sum44/2, Anti windup video 2 I actie4/1  "I actie"
  Plant H23/1 -> Continious model1/1, Sum45/2  "deltaT"
  Hold measurement2/1 -> Sum52/2, Discrete model1/1
  Sum45/1 -> Anti windup video 2 I actie4/2, Anti windup video totale command5/1, Ki7/1, Kp7/1  "error"
  Sum54/1 -> Integrator9/1
  Step17/1 -> Sum45/1
  Saturation12/1 -> Transport Delay21/1, Anti windup video totale command5/2, Sum46/1  "Na sauratie"
  Ki7/1 -> Sum48/1
  Hold U5/1 -> Plant H15/1
  Transport Delay14/1 -> Hold U5/1  "U"
  Sum51/1 -> Anti windup video totale command7/3, Sum53/2, Saturation14/1  "Voor saturatie"
  Transport Delay21/1 -> Anti windup video 2 I actie4/3, Plant H23/1  "U"
  Kp6/1 -> Scope13/2, Sum35/2
  Plant H19/1 -> Scope9/1, Sum40/2  "dTfruit"
  Sum42/1 -> Anti windup video 2 I actie3/2, Anti windup video totale command4/1, Kp6/1, Ki6/1  "error"
  Sum53/1 -> Kt5/1
  Plant H21/1 -> Scope11/1, Sum42/2  "deltaT"
  Tfruit0'2/1 -> Sum36/2
  Kp10/1 -> Sum55/1  "P actie"
  PID Controller6/1 -> Transport Delay20/1  "Voor saturatie"
  Step11/1 -> Sum38/1
  Sum48/1 -> Integrator7/1
  Step15/1 -> Sum42/1
  Transport Delay13/1 -> Plant H17/1  "U"
  Hold U4/1 -> Plant H14/1
  Saturation10/1 -> Scope16/2, Transport Delay17/1, Scope1/2  "dTset after saturation"
  Transport Delay19/1 -> Plant H21/1, Anti windup video 2 I actie3/3  "U"
  Plant H17/1 -> Scope8/1, Sum38/2  "dTfruit"
  Gain3/1 -> Scope/1, Saturation9/1  "dTset before saturation"
  Sum59/1 -> Integrator10/1
  Saturation11/1 -> Anti windup video totale command4/2, Transport Delay19/1  "Na sauratie"
  Constant3/1 -> Sum69/2
  PID Controller (Gv)2/1 -> Sum67/2, Transport Delay12/1, Delta S1/1  "Delta S"
  Kp9/1 -> Sum51/1  "P actie"
  Constant8/1 -> Sum68/1
  Transport Delay12/1 -> Plant H13/1
  Transport Delay20/1 -> Plant H22/1
  Sum37/1 -> PID Controller (Gv)2/1  "Error"
  Plant H13/1 -> Sum69/1, Hoeveel Tf veraderen1/1, Sum37/2  "deltaT"
  Plant H25/1 -> Continious model2/1, Sum71/2  "deltaT"
  Transport Delay25/1 -> Anti windup video 2 I actie clamp2/3, Plant H26/1  "U"
  Step19/1 -> Sum71/1
  Sign4/1 -> Equal5/1
  Saturation18/1 -> Rate Limiter9/1  "Na absolute sat"
  Transport Delay24/1 -> Anti windup video 2 I actie6/3, Plant H25/1  "U"
  Integrator12/1 -> Sum70/2, Anti windup video 2 I actie6/1  "I actie"
  Rate Limiter9/1 -> Anti windup video totale command9/2, Equal4/2, Transport Delay25/1  "Na sauratie"
  Sum74/1 -> Anti windup video totale command9/3, Sign5/1, Equal4/1, Saturation18/1  "Voor saturatie"
  Integrator13/1 -> Sum74/2, Anti windup video 2 I actie clamp2/1  "I actie"
  Kt8/1 -> Sum73/2
  Sum70/1 -> Anti windup video totale command8/3, Sum72/2, Saturation17/1  "Voor saturatie"
  Sign5/1 -> Equal5/2
  Saturation17/1 -> Transport Delay24/1, Anti windup video totale command8/2, Sum72/1  "Na sauratie"
  Equal4/1 -> AND2/2
  AND2/1 -> Switch2/2
  Sum71/1 -> Anti windup video 2 I actie6/2, Anti windup video totale command8/1, Ki12/1, Kp12/1  "error"
  Sum72/1 -> Kt8/1
  Equal5/1 -> AND2/1
  Ki13/1 -> Switch2/3
  Constant9/1 -> Switch2/1
  Ki12/1 -> Sum73/1
  Kp12/1 -> Sum70/1  "P actie"
  Step20/1 -> Sum75/1
  Kp13/1 -> Sum74/1  "P actie"
  Sum73/1 -> Integrator12/1
  Plant H26/1 -> Scope14/1, Sum75/2  "deltaT"
  Sum75/1 -> Anti windup video 2 I actie clamp2/2, Sign4/1, Ki13/1, Kp13/1, Anti windup video totale command9/1  "error"
  Switch2/1 -> Integrator13/1
  Step1/1 -> Sum52/1
  Sum62/1 -> Saturation16/1, Sum64/2  "U voor sat"
  Sum64/1 -> Kt7/1  "U error sat"
  Sum65/1 -> TsetOut/1
  Kt7/1 -> Integrator14/1
  Saturation16/1 -> Sum64/1, Sum65/2  "U na sat"
  Tfruitzero/1 -> Sum61/2
  TsetZero/1 -> Sum65/1
  TfruitRef/1 -> Sum61/1
  Integrator14/1 -> Sum62/2  "U anti wind"
  Sum61/1 -> Discrete PID Controller/1
  Discrete PID Controller/1 -> Sum62/1, Scope15/1
  Hold measurement5/1 -> Kt6/1
  PID Controller7/1 -> Transfer Fcn/1  "Tset"
  Sum60/1 -> PID Controller7/1  "Error Tfruit"
  Transfer Fcn/1 -> Sum60/2  "TfruitOut"
  Tfruit Ref/1 -> Sum60/1
  Integrator11/1 -> Sum39/1, Scope17/1  "I actie"
  Ki11/1 -> Integrator11/1
  Kp11/1 -> Scope18/1, Sum39/2
  Sum39/1 -> Scope1/3, Scope16/1, Saturation10/1  "dTset before saturation"
  Sum40/1 -> Scope16/3, Ki11/1, Kp11/1  "error"
  Sum49/1 -> Scope12/2, Ki8/1, Kp8/1  "error"
  Ki8/1 -> Scope19/1, Sum63/1  "I action"
  Sum63/1 -> Integrator8/1
  Plant continious/1 -> Output continious/1, Scope23/1, Continious model3/1, Sum49/2  "dTfruit continious"
  Sum50/1 -> Kt9/1
  Integrator8/1 -> Scope20/2, Sum41/2  "I action, adjusted"
  Transport Delay15/1 -> Plant continious/1  "U"
  Kp8/1 -> Scope19/3, Sum41/1, Scope20/1  "P action"
  Sum41/1 -> Scope12/3, Sum50/2, Saturation13/1  "dTset before saturation"
  Saturation13/1 -> Scope12/1, Transport Delay15/1, Sum50/1  "dTset after saturation"
  Kt9/1 -> Scope19/2, Sum63/2  "Anti-windup action"
  Integrator15/1 -> Sum66/2  "I action, adjusted"
  Sum77/1 -> "Kt "/1  "Anti-wind error"
  "Plant "/1 -> Output/1, Sum76/2  "dTfruit"
  Sum78/1 -> Integrator15/1
  "Ki "/1 -> Sum78/1  "I action"
  Sum76/1 -> "Ki "/1, "Kp "/1  "error"
  Sum66/1 -> Sum77/2, Saturation19/1  "dTset before saturation"
  "Kp "/1 -> Sum66/1  "P action"
  Time delay/1 -> "Plant "/1
  Saturation19/1 -> Time delay/1, Sum77/1  "dTset after saturation"
  "Kt "/1 -> Sum78/2  "Anti-windup action"
  Sum79/1 -> Sum81/2, Saturation20/1  "dTset before saturation"
  Anti-windup Kt/1 -> Sum79/2  "Anti-windup action"
  Saturation20/1 -> Sum92/2, Transport Delay16/1, Sum81/1  "dTset after saturation"
  Transport Delay16/1 -> Plant discrete/1  "U"
  Sum80/1 -> Zero-Order Hold2/1  "error"
  Discrete PID Controller1/1 -> Sum79/1
  Zero-Order Hold2/1 -> Discrete PID Controller1/1
  Zero-Order Hold3/1 -> Anti-windup Kt/1
  Sum81/1 -> Zero-Order Hold3/1  "Anti-wind error"
  Input continious/1 -> Sum49/1
  Sum84/1 -> Saturation21/1, Sum86/2  "Voor saturatie"
  Kt10/1 -> Sum88/2
  Sum88/1 -> Integrator16/1
  Plant H16/1 -> Hold measurement6/1  "deltaT"
  Kp14/1 -> Sum84/1  "P actie"
  Transport Delay18/1 -> Hold U6/1  "U"
  Sum82/1 -> ?
  Tfruit dat ge wilt3/1 -> Sum83/1
  Integrator16/1 -> Sum84/2  "I actie"
  Hold U6/1 -> Plant H16/1
  Sum85/1 -> Ki14/1, Kp14/1  "error"
  Tfruit5/1 -> Sum83/2
  Saturation21/1 -> Transport Delay18/1, Sum86/1, Sum87/2  "Na sauratie"
  Ki14/1 -> Sum88/1
  Hold measurement6/1 -> Sum85/2, Sum82/1, delta T discreet3/1
  Hold measurement7/1 -> Kt10/1
  Sum83/1 -> Sum85/1
  Tfruit0'3/1 -> Sum82/2
  Sum86/1 -> Hold measurement7/1
  "T Set Zero "/1 -> Sum89/1
  Sum89/1 -> T Set/1
  "T Fruit Zero "/1 -> Sum90/2
  Sum92/1 -> "T Set   "/1  "T Set"
  T Set Zero 1/1 -> Sum92/1
  Plant discrete/1 -> Sum80/2, Output discrete/1  "dTfruit"
  Sum94/1 -> "Tfruit   "/1  "T Fruit"
  T Fruit Zero 1/1 -> Sum94/2
  Input/1 -> Sum76/1
  "T Fruit Ref     "/1 -> Sum98/1
  T Set Zero 2/1 -> Sum97/1
  Sum97/1 -> T Set   1/1  "T Set"
  Zero-Order Hold5/1 -> "Anti-windup Kt    "/1
  Sum96/1 -> Scope26/1, Zero-Order Hold5/1  "Anti-wind error"
  Sum98/1 -> Zero-Order Hold4/1  "error"
  Saturation22/1 -> Scope29/1, Sum96/1  "dTset after saturation"
  "Anti-windup Kt    "/1 -> Zero-Order Hold7/1  "Anti-windup action"
  Sum91/1 -> Scope27/1, Sum96/2, Saturation22/1  "dTset before saturation"
  Zero-Order Hold4/1 -> Discrete PID Controller2/1
  "T Fruit Zero     "/1 -> Sum98/2
  Discrete PID Controller2/1 -> Zero-Order Hold6/1
  Zero-Order Hold6/1 -> Sum91/1
  Zero-Order Hold7/1 -> Scope25/1, Sum91/2  "Anti-windup action"
  Input discrete/1 -> Sum80/1
  T Fruit Zero  2/1 -> Sum102/2
  Sum101/1 -> T Set   2/1  "T Set"
  Transport Delay22/1 -> Plant discrete1/1  "U"
  Saturation23/1 -> Sum101/2, Transport Delay22/1, Sum100/1  "dTset after saturation"
  Plant discrete1/1 -> Sum94/1, Sum99/2, Scope34/1  "dTfruit"
  T Set Zero 3/1 -> Sum101/1
  T Fruit Ref2/1 -> Sum102/1
  Sum100/1 -> Scope31/1, Zero-Order Hold9/1  "Anti-wind error"
  Zero-Order Hold9/1 -> Anti-windup Kt1/1
  Zero-Order Hold8/1 -> Discrete PID Controller3/1
  Discrete PID Controller3/1 -> Sum95/1
  Anti-windup Kt1/1 -> Scope33/1, Sum95/2  "Anti-windup action"
  Sum95/1 -> Scope32/1, Sum100/2, Saturation23/1  "dTset before saturation"
  Sum99/1 -> Zero-Order Hold8/1  "error"
  Sum102/1 -> Sum99/1
  Anti-windup Kt2/1 -> Scope24/1, Sum106/2  "Anti-windup action"
  Sum107/1 -> Zero-Order Hold10/1  "error"
  T Set Zero 4/1 -> Sum103/1
  Zero-Order Hold11/1 -> Anti-windup Kt2/1
  Saturation24/1 -> Sum103/2, Transport Delay26/1, Sum93/1  "dTset after saturation"
  Plant discrete2/1 -> Sum105/1, Sum107/2, Scope30/1  "dTfruit"
  T Fruit Ref1/1 -> Sum104/1
  Zero-Order Hold10/1 -> Discrete PID Controller4/1
  Sum93/1 -> Scope21/1, Zero-Order Hold11/1  "Anti-wind error"
  Discrete PID Controller4/1 -> Sum106/1
  Sum106/1 -> Scope22/1, Sum93/2, Saturation24/1  "dTset before saturation"
  Sum103/1 -> T Set   3/1  "T Set"
  Sum104/1 -> Sum107/1
  Transport Delay26/1 -> Plant discrete2/1  "U"
  Sum105/1 -> Tfruit   1/1  "T Fruit"
  T Fruit Zero  1/1 -> Sum104/2
  T Fruit Zero 2/1 -> Sum105/2
  T Fruit Zero 3/1 -> Sum109/2
  T Set Zero 5/1 -> Sum108/1
  Sum108/1 -> Scope37/1, T Set   4/1  "T Set"
  Sum109/1 -> Scope37/2, Tfruit   2/1  "T Fruit"
  Transport Delay27/1 -> Plant discrete3/1  "U"
  Plant discrete3/1 -> Sum109/1, Scope35/1  "dTfruit"
  Transport Delay28/1 -> Plant discrete4/1  "U"
  Sum110/1 -> Scope38/1, T Set   5/1  "T Set"
  Sum111/1 -> Scope38/2, Tfruit   3/1  "T Fruit"
  T Fruit Zero 4/1 -> Sum111/2
  Plant discrete4/1 -> Sum111/1, Scope36/1  "dTfruit"
  T Set Zero 6/1 -> Sum110/1
  Step -0.0247/1 -> Sum108/2, Transport Delay27/1  "dTset"
  -1.75°C1/1(Signal 1) -> Sum110/2, Transport Delay28/1  "dTset"
